simulink model "RADTRANS002"  (R2020b)
(part 2 of 7)

      |     % Цикл начинаем с 2, так как 1-й элемент в списке - это сама папка подсистемы
      |     for i = 2:length(internalBlocks)
      |         oldName = get_param(internalBlocks{i}, 'Name');
      |         % Ищем цифру в конце имени и меняем на новую
      |         newName = regexprep(oldName, '\d+$', newNum);
      | 
      |         % Если имя изменилось, применяем его
      |         if ~strcmp(oldName, newName)
      |             try
      |                 set_param(internalBlocks{i}, 'Name', newName);
      |             catch
      |                 % Игнорируем ошибку, если вдруг такое имя уже случайно есть
      |             end
      |         end
      |     end
      | end
  M_OUT_Завод_4_2 : Subsystem
      settings: CopyFcn=|
      | % Получаем путь и имя нового (только что скопированного) блока
      | blockPath = gcb;
      | blockName = get_param(blockPath, 'Name');
      | 
      | % Ищем число в названии самой подсистемы (например, берем "2" из "Measure_2")
      | numStr = regexp(blockName, '\d+', 'match');
      | 
      | if ~isempty(numStr)
      |     newNum = numStr{end}; % Берем последнее найденное число
      | 
      |     % --- 1. Обновляем скрытые теги в Goto и From (радиочастоты) ---
      |     gotos = find_system(blockPath, 'LookUnderMasks', 'on', 'BlockType', 'Goto');
      |     froms = find_system(blockPath, 'LookUnderMasks', 'on', 'BlockType', 'From');
      | 
      |     for i = 1:length(gotos)
      |         oldTag = get_param(gotos{i}, 'GotoTag');
      |         set_param(gotos{i}, 'GotoTag', regexprep(oldTag, '\d+$', newNum));
      |     end
      |     for i = 1:length(froms)
      |         oldTag = get_param(froms{i}, 'GotoTag');
      |         set_param(froms{i}, 'GotoTag', regexprep(oldTag, '\d+$', newNum));
      |     end
      | 
      |     % --- 2. ПЕРЕИМЕНОВЫВАЕМ САМИ БЛОКИ (визуальные надписи UI0 -> UI1 и т.д.) ---
      |     % Ищем все элементы только внутри этой подсистемы
      |     internalBlocks = find_system(blockPath, 'SearchDepth', 1, 'LookUnderMasks', 'on');
      | 
      |     % Цикл начинаем с 2, так как 1-й элемент в списке - это сама папка подсистемы
      |     for i = 2:length(internalBlocks)
      |         oldName = get_param(internalBlocks{i}, 'Name');
      |         % Ищем цифру в конце имени и меняем на новую
      |         newName = regexprep(oldName, '\d+$', newNum);
      | 
      |         % Если имя изменилось, применяем его
      |         if ~strcmp(oldName, newName)
      |             try
      |                 set_param(internalBlocks{i}, 'Name', newName);
      |             catch
      |                 % Игнорируем ошибку, если вдруг такое имя уже случайно есть
      |             end
      |         end
      |     end
      | end
  M_OUT_Завод_5_1 : Subsystem
      settings: CopyFcn=|
      | % Получаем путь и имя нового (только что скопированного) блока
      | blockPath = gcb;
      | blockName = get_param(blockPath, 'Name');
      | 
      | % Ищем число в названии самой подсистемы (например, берем "2" из "Measure_2")
      | numStr = regexp(blockName, '\d+', 'match');
      | 
      | if ~isempty(numStr)
      |     newNum = numStr{end}; % Берем последнее найденное число
      | 
      |     % --- 1. Обновляем скрытые теги в Goto и From (радиочастоты) ---
      |     gotos = find_system(blockPath, 'LookUnderMasks', 'on', 'BlockType', 'Goto');
      |     froms = find_system(blockPath, 'LookUnderMasks', 'on', 'BlockType', 'From');
      | 
      |     for i = 1:length(gotos)
      |         oldTag = get_param(gotos{i}, 'GotoTag');
      |         set_param(gotos{i}, 'GotoTag', regexprep(oldTag, '\d+$', newNum));
      |     end
      |     for i = 1:length(froms)
      |         oldTag = get_param(froms{i}, 'GotoTag');
      |         set_param(froms{i}, 'GotoTag', regexprep(oldTag, '\d+$', newNum));
      |     end
      | 
      |     % --- 2. ПЕРЕИМЕНОВЫВАЕМ САМИ БЛОКИ (визуальные надписи UI0 -> UI1 и т.д.) ---
      |     % Ищем все элементы только внутри этой подсистемы
      |     internalBlocks = find_system(blockPath, 'SearchDepth', 1, 'LookUnderMasks', 'on');
      | 
      |     % Цикл начинаем с 2, так как 1-й элемент в списке - это сама папка подсистемы
      |     for i = 2:length(internalBlocks)
      |         oldName = get_param(internalBlocks{i}, 'Name');
      |         % Ищем цифру в конце имени и меняем на новую
      |         newName = regexprep(oldName, '\d+$', newNum);
      | 
      |         % Если имя изменилось, применяем его
      |         if ~strcmp(oldName, newName)
      |             try
      |                 set_param(internalBlocks{i}, 'Name', newName);
      |             catch
      |                 % Игнорируем ошибку, если вдруг такое имя уже случайно есть
      |             end
      |         end
      |     end
      | end
  M_OUT_Завод_5_2 : Subsystem
      settings: CopyFcn=|
      | % Получаем путь и имя нового (только что скопированного) блока
      | blockPath = gcb;
      | blockName = get_param(blockPath, 'Name');
      | 
      | % Ищем число в названии самой подсистемы (например, берем "2" из "Measure_2")
      | numStr = regexp(blockName, '\d+', 'match');
      | 
      | if ~isempty(numStr)
      |     newNum = numStr{end}; % Берем последнее найденное число
      | 
      |     % --- 1. Обновляем скрытые теги в Goto и From (радиочастоты) ---
      |     gotos = find_system(blockPath, 'LookUnderMasks', 'on', 'BlockType', 'Goto');
      |     froms = find_system(blockPath, 'LookUnderMasks', 'on', 'BlockType', 'From');
      | 
      |     for i = 1:length(gotos)
      |         oldTag = get_param(gotos{i}, 'GotoTag');
      |         set_param(gotos{i}, 'GotoTag', regexprep(oldTag, '\d+$', newNum));
      |     end
      |     for i = 1:length(froms)
      |         oldTag = get_param(froms{i}, 'GotoTag');
      |         set_param(froms{i}, 'GotoTag', regexprep(oldTag, '\d+$', newNum));
      |     end
      | 
      |     % --- 2. ПЕРЕИМЕНОВЫВАЕМ САМИ БЛОКИ (визуальные надписи UI0 -> UI1 и т.д.) ---
      |     % Ищем все элементы только внутри этой подсистемы
      |     internalBlocks = find_system(blockPath, 'SearchDepth', 1, 'LookUnderMasks', 'on');
      | 
      |     % Цикл начинаем с 2, так как 1-й элемент в списке - это сама папка подсистемы
      |     for i = 2:length(internalBlocks)
      |         oldName = get_param(internalBlocks{i}, 'Name');
      |         % Ищем цифру в конце имени и меняем на новую
      |         newName = regexprep(oldName, '\d+$', newNum);
      | 
      |         % Если имя изменилось, применяем его
      |         if ~strcmp(oldName, newName)
      |             try
      |                 set_param(internalBlocks{i}, 'Name', newName);
      |             catch
      |                 % Игнорируем ошибку, если вдруг такое имя уже случайно есть
      |             end
      |         end
      |     end
      | end
  M_OUT_Завод_6_1 : Subsystem
      settings: CopyFcn=|
      | % Получаем путь и имя нового (только что скопированного) блока
      | blockPath = gcb;
      | blockName = get_param(blockPath, 'Name');
      | 
      | % Ищем число в названии самой подсистемы (например, берем "2" из "Measure_2")
      | numStr = regexp(blockName, '\d+', 'match');
      | 
      | if ~isempty(numStr)
      |     newNum = numStr{end}; % Берем последнее найденное число
      | 
      |     % --- 1. Обновляем скрытые теги в Goto и From (радиочастоты) ---
      |     gotos = find_system(blockPath, 'LookUnderMasks', 'on', 'BlockType', 'Goto');
      |     froms = find_system(blockPath, 'LookUnderMasks', 'on', 'BlockType', 'From');
      | 
      |     for i = 1:length(gotos)
      |         oldTag = get_param(gotos{i}, 'GotoTag');
      |         set_param(gotos{i}, 'GotoTag', regexprep(oldTag, '\d+$', newNum));
      |     end
      |     for i = 1:length(froms)
      |         oldTag = get_param(froms{i}, 'GotoTag');
      |         set_param(froms{i}, 'GotoTag', regexprep(oldTag, '\d+$', newNum));
      |     end
      | 
      |     % --- 2. ПЕРЕИМЕНОВЫВАЕМ САМИ БЛОКИ (визуальные надписи UI0 -> UI1 и т.д.) ---
      |     % Ищем все элементы только внутри этой подсистемы
      |     internalBlocks = find_system(blockPath, 'SearchDepth', 1, 'LookUnderMasks', 'on');
      | 
      |     % Цикл начинаем с 2, так как 1-й элемент в списке - это сама папка подсистемы
      |     for i = 2:length(internalBlocks)
      |         oldName = get_param(internalBlocks{i}, 'Name');
      |         % Ищем цифру в конце имени и меняем на новую
      |         newName = regexprep(oldName, '\d+$', newNum);
      | 
      |         % Если имя изменилось, применяем его
      |         if ~strcmp(oldName, newName)
      |             try
      |                 set_param(internalBlocks{i}, 'Name', newName);
      |             catch
      |                 % Игнорируем ошибку, если вдруг такое имя уже случайно есть
      |             end
      |         end
      |     end
      | end
  M_OUT_Завод_6_2 : Subsystem
      settings: CopyFcn=|
      | % Получаем путь и имя нового (только что скопированного) блока
      | blockPath = gcb;
      | blockName = get_param(blockPath, 'Name');
      | 
      | % Ищем число в названии самой подсистемы (например, берем "2" из "Measure_2")
      | numStr = regexp(blockName, '\d+', 'match');
      | 
      | if ~isempty(numStr)
      |     newNum = numStr{end}; % Берем последнее найденное число
      | 
      |     % --- 1. Обновляем скрытые теги в Goto и From (радиочастоты) ---
      |     gotos = find_system(blockPath, 'LookUnderMasks', 'on', 'BlockType', 'Goto');
      |     froms = find_system(blockPath, 'LookUnderMasks', 'on', 'BlockType', 'From');
      | 
      |     for i = 1:length(gotos)
      |         oldTag = get_param(gotos{i}, 'GotoTag');
      |         set_param(gotos{i}, 'GotoTag', regexprep(oldTag, '\d+$', newNum));
      |     end
      |     for i = 1:length(froms)
      |         oldTag = get_param(froms{i}, 'GotoTag');
      |         set_param(froms{i}, 'GotoTag', regexprep(oldTag, '\d+$', newNum));
      |     end
      | 
      |     % --- 2. ПЕРЕИМЕНОВЫВАЕМ САМИ БЛОКИ (визуальные надписи UI0 -> UI1 и т.д.) ---
      |     % Ищем все элементы только внутри этой подсистемы
      |     internalBlocks = find_system(blockPath, 'SearchDepth', 1, 'LookUnderMasks', 'on');
      | 
      |     % Цикл начинаем с 2, так как 1-й элемент в списке - это сама папка подсистемы
      |     for i = 2:length(internalBlocks)
      |         oldName = get_param(internalBlocks{i}, 'Name');
      |         % Ищем цифру в конце имени и меняем на новую
      |         newName = regexprep(oldName, '\d+$', newNum);
      | 
      |         % Если имя изменилось, применяем его
      |         if ~strcmp(oldName, newName)
      |             try
      |                 set_param(internalBlocks{i}, 'Name', newName);
      |             catch
      |                 % Игнорируем ошибку, если вдруг такое имя уже случайно есть
      |             end
      |         end
      |     end
      | end
  Powergui : powerlib/powergui  Priority=1  SimulationMode=Discrete  SampleTime=Ts_powergui  frequency=60  Iterations=50  frequencyindice=50  Pbase=100e6  ErrMax=1e-4  UnitsV=kV  UnitsW=MW  buscounter=0  FunctionMessages=off  echomessages=off  EnableUseOfTLC=off  CurrentSourceSwitches=off  DisableSnubberDevices=off  DisableRonSwitches=off  DisableVfSwitches=off  DisplayEquations=off  AutomaticDiscreteSolvers=off  SolverType=Tustin/Backward Euler (TBE)  Interpol=off  ExternalGateDelay=off  methode=off  Ts=100  x0status=blocks  SPID=on  SwTol=0  HookPort=off  NonlinearTolerance=1e-4  nMaxIteration=100  ContinueOnMaxIteration=off  RestoreLinks=warning  ResistiveCurrentMeasurement=off  Frange=[0:2:500]  Ylog=off  Xlog=on  ShowGrid=off  save=off  variable=ZData  structure=0  ZoomFFT=off  StartTime=0.0  cycles=1  DisplayStyle=1  fundamental=60  FreqAxis=off  MaxFrequency=1000  frequencyindicesteady=1  RmsSteady=1  display=off
  Источник_220кВ : powerlib/Electrical Sources/Three-Phase Source  InternalConnection=Yg  VoltagePhases=off  Voltage=Sys_V_net_kV * 1e3  PhaseAngle=0  Voltage_phases=[25e3 25e3 25e3]/sqrt(3)  PhaseAngles_phases=[0 -120 +120]  Frequency=Sys_f_Hz  NonIdealSource=on  SpecifyImpedance=off  Resistance=0.8929  Inductance=16.58e-3  ShortCircuitLevel=Sys_S_sc_VA  BaseVoltage=Sys_V_net_kV * 1e3  XRratio=7  BusType=swing  Pref=10e3  Qref=0  Prefabc=[10e3, 10e3, 10e3]  Qrefabc=[0, 0, 0]  Qmin=-inf  Qmax=inf
  Линия_110кВ_Район_{1..6} (6 alike) : powerlib/Elements/Three-Phase PI Section Line  LConnTagsString=a|b|c  RConnTagsString=A|B|C  Length=1  Frequency=Sys_f_Hz  Resistances=[Line_110_R, Line_110_R*3]  Inductances=[Line_110_L, Line_110_L*3]  Capacitances=[Line_110_C, Line_110_C]
  Линия_Город_1_{1..4} (4 alike) : powerlib/Elements/Three-Phase PI Section Line  LConnTagsString=a|b|c  RConnTagsString=A|B|C  Length=1  Frequency=Sys_f_Hz  Resistances=[Line_6_R, Line_6_R*3]  Inductances=[Line_6_L, Line_6_L*3]  Capacitances=[1e-9, 1e-9]
  Линия_Город_2_{1..4} (4 alike) : powerlib/Elements/Three-Phase PI Section Line  LConnTagsString=a|b|c  RConnTagsString=A|B|C  Length=1  Frequency=Sys_f_Hz  Resistances=[Line_6_R, Line_6_R*3]  Inductances=[Line_6_L, Line_6_L*3]  Capacitances=[1e-9, 1e-9]
  Линия_Город_3_{1..4} (4 alike) : powerlib/Elements/Three-Phase PI Section Line  LConnTagsString=a|b|c  RConnTagsString=A|B|C  Length=1  Frequency=Sys_f_Hz  Resistances=[Line_6_R, Line_6_R*3]  Inductances=[Line_6_L, Line_6_L*3]  Capacitances=[1e-9, 1e-9]
  Линия_Город_4_{1..4} (4 alike) : powerlib/Elements/Three-Phase PI Section Line  LConnTagsString=a|b|c  RConnTagsString=A|B|C  Length=1  Frequency=Sys_f_Hz  Resistances=[Line_6_R, Line_6_R*3]  Inductances=[Line_6_L, Line_6_L*3]  Capacitances=[1e-9, 1e-9]
  Линия_Город_5_{1..4} (4 alike) : powerlib/Elements/Three-Phase PI Section Line  LConnTagsString=a|b|c  RConnTagsString=A|B|C  Length=1  Frequency=Sys_f_Hz  Resistances=[Line_6_R, Line_6_R*3]  Inductances=[Line_6_L, Line_6_L*3]  Capacitances=[1e-9, 1e-9]
  Линия_Город_6_{1..4} (4 alike) : powerlib/Elements/Three-Phase PI Section Line  LConnTagsString=a|b|c  RConnTagsString=A|B|C  Length=1  Frequency=Sys_f_Hz  Resistances=[Line_6_R, Line_6_R*3]  Inductances=[Line_6_L, Line_6_L*3]  Capacitances=[1e-9, 1e-9]
  Линия_Завод_1_1 : powerlib/Elements/Three-Phase PI Section Line  LConnTagsString=a|b|c  RConnTagsString=A|B|C  Length=1  Frequency=Sys_f_Hz  Resistances=[Line_35_R, Line_35_R*3]  Inductances=[Line_35_L, Line_35_L*3]  Capacitances=[Line_35_C, Line_35_C]
  Линия_Завод_1_2 : powerlib/Elements/Three-Phase PI Section Line  LConnTagsString=a|b|c  RConnTagsString=A|B|C  Length=1  Frequency=Sys_f_Hz  Resistances=[Line_35_R, Line_35_R*3]  Inductances=[Line_35_L, Line_35_L*3]  Capacitances=[Line_35_C, Line_35_C]
  Линия_Завод_2_1 : powerlib/Elements/Three-Phase PI Section Line  LConnTagsString=a|b|c  RConnTagsString=A|B|C  Length=1  Frequency=Sys_f_Hz  Resistances=[Line_35_R, Line_35_R*3]  Inductances=[Line_35_L, Line_35_L*3]  Capacitances=[Line_35_C, Line_35_C]
  Линия_Завод_2_2 : powerlib/Elements/Three-Phase PI Section Line  LConnTagsString=a|b|c  RConnTagsString=A|B|C  Length=1  Frequency=Sys_f_Hz  Resistances=[Line_35_R, Line_35_R*3]  Inductances=[Line_35_L, Line_35_L*3]  Capacitances=[Line_35_C, Line_35_C]
  Линия_Завод_3_1 : powerlib/Elements/Three-Phase PI Section Line  LConnTagsString=a|b|c  RConnTagsString=A|B|C  Length=1  Frequency=Sys_f_Hz  Resistances=[Line_35_R, Line_35_R*3]  Inductances=[Line_35_L, Line_35_L*3]  Capacitances=[Line_35_C, Line_35_C]
  Линия_Завод_3_2 : powerlib/Elements/Three-Phase PI Section Line  LConnTagsString=a|b|c  RConnTagsString=A|B|C  Length=1  Frequency=Sys_f_Hz  Resistances=[Line_35_R, Line_35_R*3]  Inductances=[Line_35_L, Line_35_L*3]  Capacitances=[Line_35_C, Line_35_C]
  Линия_Завод_4_1 : powerlib/Elements/Three-Phase PI Section Line  LConnTagsString=a|b|c  RConnTagsString=A|B|C  Length=1  Frequency=Sys_f_Hz  Resistances=[Line_35_R, Line_35_R*3]  Inductances=[Line_35_L, Line_35_L*3]  Capacitances=[Line_35_C, Line_35_C]
  Линия_Завод_4_2 : powerlib/Elements/Three-Phase PI Section Line  LConnTagsString=a|b|c  RConnTagsString=A|B|C  Length=1  Frequency=Sys_f_Hz  Resistances=[Line_35_R, Line_35_R*3]  Inductances=[Line_35_L, Line_35_L*3]  Capacitances=[Line_35_C, Line_35_C]
  Линия_Завод_5_1 : powerlib/Elements/Three-Phase PI Section Line  LConnTagsString=a|b|c  RConnTagsString=A|B|C  Length=1  Frequency=Sys_f_Hz  Resistances=[Line_35_R, Line_35_R*3]  Inductances=[Line_35_L, Line_35_L*3]  Capacitances=[Line_35_C, Line_35_C]
  Линия_Завод_5_2 : powerlib/Elements/Three-Phase PI Section Line  LConnTagsString=a|b|c  RConnTagsString=A|B|C  Length=1  Frequency=Sys_f_Hz  Resistances=[Line_35_R, Line_35_R*3]  Inductances=[Line_35_L, Line_35_L*3]  Capacitances=[Line_35_C, Line_35_C]
  Линия_Завод_6_1 : powerlib/Elements/Three-Phase PI Section Line  LConnTagsString=a|b|c  RConnTagsString=A|B|C  Length=1  Frequency=Sys_f_Hz  Resistances=[Line_35_R, Line_35_R*3]  Inductances=[Line_35_L, Line_35_L*3]  Capacitances=[Line_35_C, Line_35_C]
  Линия_Завод_6_2 : powerlib/Elements/Three-Phase PI Section Line  LConnTagsString=a|b|c  RConnTagsString=A|B|C  Length=1  Frequency=Sys_f_Hz  Resistances=[Line_35_R, Line_35_R*3]  Inductances=[Line_35_L, Line_35_L*3]  Capacitances=[Line_35_C, Line_35_C]
  Магистраль_220кВ : powerlib/Elements/Three-Phase PI Section Line  LConnTagsString=a|b|c  RConnTagsString=A|B|C  Length=1  Frequency=Sys_f_Hz  Resistances=[Line_220_R, Line_220_R*3]  Inductances=[Line_220_L, Line_220_L*3]  Capacitances=[Line_220_C, Line_220_C]
  Нагрузка_Город_1_{1..4} (4 alike) : powerlib/Elements/Three-Phase Series RLC Load  LConnTagsString=A|B|C  Configuration=Y (grounded)  NominalVoltage=Tr_6_04_V_LV_kV*1e3  Vabc=[1e3 1e3 1e3]  Vabcp=[1e3 1e3 1e3]  NominalFrequency=Sys_f_Hz  UnbalancedPower=off  ActivePower=Load_City_P  InductivePower=Load_City_Q  CapacitivePower=0  Pabc=[10e3 9e3 11e3]  QLabc=[100 90 110]  QCabc=[100 90 110]  Pabcp=[10e3 9e3 11e3]  QLabcp=[100 90 110]  QCabcp=[100 90 110]  Measurements=None  LoadType=constant Z
  Нагрузка_Город_2_{1..4} (4 alike) : powerlib/Elements/Three-Phase Series RLC Load  LConnTagsString=A|B|C  Configuration=Y (grounded)  NominalVoltage=Tr_6_04_V_LV_kV*1e3  Vabc=[1e3 1e3 1e3]  Vabcp=[1e3 1e3 1e3]  NominalFrequency=Sys_f_Hz  UnbalancedPower=off  ActivePower=Load_City_P  InductivePower=Load_City_Q  CapacitivePower=0  Pabc=[10e3 9e3 11e3]  QLabc=[100 90 110]  QCabc=[100 90 110]  Pabcp=[10e3 9e3 11e3]  QLabcp=[100 90 110]  QCabcp=[100 90 110]  Measurements=None  LoadType=constant Z
  Нагрузка_Город_3_{1..4} (4 alike) : powerlib/Elements/Three-Phase Series RLC Load  LConnTagsString=A|B|C  Configuration=Y (grounded)  NominalVoltage=Tr_6_04_V_LV_kV*1e3  Vabc=[1e3 1e3 1e3]  Vabcp=[1e3 1e3 1e3]  NominalFrequency=Sys_f_Hz  UnbalancedPower=off  ActivePower=Load_City_P  InductivePower=Load_City_Q  CapacitivePower=0  Pabc=[10e3 9e3 11e3]  QLabc=[100 90 110]  QCabc=[100 90 110]  Pabcp=[10e3 9e3 11e3]  QLabcp=[100 90 110]  QCabcp=[100 90 110]  Measurements=None  LoadType=constant Z
  Нагрузка_Город_4_{1..4} (4 alike) : powerlib/Elements/Three-Phase Series RLC Load  LConnTagsString=A|B|C  Configuration=Y (grounded)  NominalVoltage=Tr_6_04_V_LV_kV*1e3  Vabc=[1e3 1e3 1e3]  Vabcp=[1e3 1e3 1e3]  NominalFrequency=Sys_f_Hz  UnbalancedPower=off  ActivePower=Load_City_P  InductivePower=Load_City_Q  CapacitivePower=0  Pabc=[10e3 9e3 11e3]  QLabc=[100 90 110]  QCabc=[100 90 110]  Pabcp=[10e3 9e3 11e3]  QLabcp=[100 90 110]  QCabcp=[100 90 110]  Measurements=None  LoadType=constant Z
  Нагрузка_Город_5_{1..4} (4 alike) : powerlib/Elements/Three-Phase Series RLC Load  LConnTagsString=A|B|C  Configuration=Y (grounded)  NominalVoltage=Tr_6_04_V_LV_kV*1e3  Vabc=[1e3 1e3 1e3]  Vabcp=[1e3 1e3 1e3]  NominalFrequency=Sys_f_Hz  UnbalancedPower=off  ActivePower=Load_City_P  InductivePower=Load_City_Q  CapacitivePower=0  Pabc=[10e3 9e3 11e3]  QLabc=[100 90 110]  QCabc=[100 90 110]  Pabcp=[10e3 9e3 11e3]  QLabcp=[100 90 110]  QCabcp=[100 90 110]  Measurements=None  LoadType=constant Z
  Нагрузка_Город_6_{1..4} (4 alike) : powerlib/Elements/Three-Phase Series RLC Load  LConnTagsString=A|B|C  Configuration=Y (grounded)  NominalVoltage=Tr_6_04_V_LV_kV*1e3  Vabc=[1e3 1e3 1e3]  Vabcp=[1e3 1e3 1e3]  NominalFrequency=Sys_f_Hz  UnbalancedPower=off  ActivePower=Load_City_P  InductivePower=Load_City_Q  CapacitivePower=0  Pabc=[10e3 9e3 11e3]  QLabc=[100 90 110]  QCabc=[100 90 110]  Pabcp=[10e3 9e3 11e3]  QLabcp=[100 90 110]  QCabcp=[100 90 110]  Measurements=None  LoadType=constant Z
  Нагрузка_Завод_1_1 : powerlib/Elements/Three-Phase Series RLC Load  LConnTagsString=A|B|C  Configuration=Y (grounded)  NominalVoltage=Tr_35_04_V_LV_kV*1e3  Vabc=[1e3 1e3 1e3]  Vabcp=[1e3 1e3 1e3]  NominalFrequency=Sys_f_Hz  UnbalancedPower=off  ActivePower=Load_Factory_P  InductivePower=Load_Factory_Q  CapacitivePower=0  Pabc=[10e3 9e3 11e3]  QLabc=[100 90 110]  QCabc=[100 90 110]  Pabcp=[10e3 9e3 11e3]  QLabcp=[100 90 110]  QCabcp=[100 90 110]  Measurements=None  LoadType=constant Z
  Нагрузка_Завод_1_2 : powerlib/Elements/Three-Phase Series RLC Load  LConnTagsString=A|B|C  Configuration=Y (grounded)  NominalVoltage=Tr_35_04_V_LV_kV*1e3  Vabc=[1e3 1e3 1e3]  Vabcp=[1e3 1e3 1e3]  NominalFrequency=Sys_f_Hz  UnbalancedPower=off  ActivePower=Load_Factory_P  InductivePower=Load_Factory_Q  CapacitivePower=0  Pabc=[10e3 9e3 11e3]  QLabc=[100 90 110]  QCabc=[100 90 110]  Pabcp=[10e3 9e3 11e3]  QLabcp=[100 90 110]  QCabcp=[100 90 110]  Measurements=None  LoadType=constant Z
  Нагрузка_Завод_2_1 : powerlib/Elements/Three-Phase Series RLC Load  LConnTagsString=A|B|C  Configuration=Y (grounded)  NominalVoltage=Tr_35_04_V_LV_kV*1e3  Vabc=[1e3 1e3 1e3]  Vabcp=[1e3 1e3 1e3]  NominalFrequency=Sys_f_Hz  UnbalancedPower=off  ActivePower=Load_Factory_P  InductivePower=Load_Factory_Q  CapacitivePower=0  Pabc=[10e3 9e3 11e3]  QLabc=[100 90 110]  QCabc=[100 90 110]  Pabcp=[10e3 9e3 11e3]  QLabcp=[100 90 110]  QCabcp=[100 90 110]  Measurements=None  LoadType=constant Z
  Нагрузка_Завод_2_2 : powerlib/Elements/Three-Phase Series RLC Load  LConnTagsString=A|B|C  Configuration=Y (grounded)  NominalVoltage=Tr_35_04_V_LV_kV*1e3  Vabc=[1e3 1e3 1e3]  Vabcp=[1e3 1e3 1e3]  NominalFrequency=Sys_f_Hz  UnbalancedPower=off  ActivePower=Load_Factory_P  InductivePower=Load_Factory_Q  CapacitivePower=0  Pabc=[10e3 9e3 11e3]  QLabc=[100 90 110]  QCabc=[100 90 110]  Pabcp=[10e3 9e3 11e3]  QLabcp=[100 90 110]  QCabcp=[100 90 110]  Measurements=None  LoadType=constant Z
  Нагрузка_Завод_3_1 : powerlib/Elements/Three-Phase Series RLC Load  LConnTagsString=A|B|C  Configuration=Y (grounded)  NominalVoltage=Tr_35_04_V_LV_kV*1e3  Vabc=[1e3 1e3 1e3]  Vabcp=[1e3 1e3 1e3]  NominalFrequency=Sys_f_Hz  UnbalancedPower=off  ActivePower=Load_Factory_P  InductivePower=Load_Factory_Q  CapacitivePower=0  Pabc=[10e3 9e3 11e3]  QLabc=[100 90 110]  QCabc=[100 90 110]  Pabcp=[10e3 9e3 11e3]  QLabcp=[100 90 110]  QCabcp=[100 90 110]  Measurements=None  LoadType=constant Z
  Нагрузка_Завод_3_2 : powerlib/Elements/Three-Phase Series RLC Load  LConnTagsString=A|B|C  Configuration=Y (grounded)  NominalVoltage=Tr_35_04_V_LV_kV*1e3  Vabc=[1e3 1e3 1e3]  Vabcp=[1e3 1e3 1e3]  NominalFrequency=Sys_f_Hz  UnbalancedPower=off  ActivePower=Load_Factory_P  InductivePower=Load_Factory_Q  CapacitivePower=0  Pabc=[10e3 9e3 11e3]  QLabc=[100 90 110]  QCabc=[100 90 110]  Pabcp=[10e3 9e3 11e3]  QLabcp=[100 90 110]  QCabcp=[100 90 110]  Measurements=None  LoadType=constant Z
  Нагрузка_Завод_4_1 : powerlib/Elements/Three-Phase Series RLC Load  LConnTagsString=A|B|C  Configuration=Y (grounded)  NominalVoltage=Tr_35_04_V_LV_kV*1e3  Vabc=[1e3 1e3 1e3]  Vabcp=[1e3 1e3 1e3]  NominalFrequency=Sys_f_Hz  UnbalancedPower=off  ActivePower=Load_Factory_P  InductivePower=Load_Factory_Q  CapacitivePower=0  Pabc=[10e3 9e3 11e3]  QLabc=[100 90 110]  QCabc=[100 90 110]  Pabcp=[10e3 9e3 11e3]  QLabcp=[100 90 110]  QCabcp=[100 90 110]  Measurements=None  LoadType=constant Z
  Нагрузка_Завод_4_2 : powerlib/Elements/Three-Phase Series RLC Load  LConnTagsString=A|B|C  Configuration=Y (grounded)  NominalVoltage=Tr_35_04_V_LV_kV*1e3  Vabc=[1e3 1e3 1e3]  Vabcp=[1e3 1e3 1e3]  NominalFrequency=Sys_f_Hz  UnbalancedPower=off  ActivePower=Load_Factory_P  InductivePower=Load_Factory_Q  CapacitivePower=0  Pabc=[10e3 9e3 11e3]  QLabc=[100 90 110]  QCabc=[100 90 110]  Pabcp=[10e3 9e3 11e3]  QLabcp=[100 90 110]  QCabcp=[100 90 110]  Measurements=None  LoadType=constant Z
  Нагрузка_Завод_5_1 : powerlib/Elements/Three-Phase Series RLC Load  LConnTagsString=A|B|C  Configuration=Y (grounded)  NominalVoltage=Tr_35_04_V_LV_kV*1e3  Vabc=[1e3 1e3 1e3]  Vabcp=[1e3 1e3 1e3]  NominalFrequency=Sys_f_Hz  UnbalancedPower=off  ActivePower=Load_Factory_P  InductivePower=Load_Factory_Q  CapacitivePower=0  Pabc=[10e3 9e3 11e3]  QLabc=[100 90 110]  QCabc=[100 90 110]  Pabcp=[10e3 9e3 11e3]  QLabcp=[100 90 110]  QCabcp=[100 90 110]  Measurements=None  LoadType=constant Z
  Нагрузка_Завод_5_2 : powerlib/Elements/Three-Phase Series RLC Load  LConnTagsString=A|B|C  Configuration=Y (grounded)  NominalVoltage=Tr_35_04_V_LV_kV*1e3  Vabc=[1e3 1e3 1e3]  Vabcp=[1e3 1e3 1e3]  NominalFrequency=Sys_f_Hz  UnbalancedPower=off  ActivePower=Load_Factory_P  InductivePower=Load_Factory_Q  CapacitivePower=0  Pabc=[10e3 9e3 11e3]  QLabc=[100 90 110]  QCabc=[100 90 110]  Pabcp=[10e3 9e3 11e3]  QLabcp=[100 90 110]  QCabcp=[100 90 110]  Measurements=None  LoadType=constant Z
  Нагрузка_Завод_6_1 : powerlib/Elements/Three-Phase Series RLC Load  LConnTagsString=A|B|C  Configuration=Y (grounded)  NominalVoltage=Tr_35_04_V_LV_kV*1e3  Vabc=[1e3 1e3 1e3]  Vabcp=[1e3 1e3 1e3]  NominalFrequency=Sys_f_Hz  UnbalancedPower=off  ActivePower=Load_Factory_P  InductivePower=Load_Factory_Q  CapacitivePower=0  Pabc=[10e3 9e3 11e3]  QLabc=[100 90 110]  QCabc=[100 90 110]  Pabcp=[10e3 9e3 11e3]  QLabcp=[100 90 110]  QCabcp=[100 90 110]  Measurements=None  LoadType=constant Z
  Нагрузка_Завод_6_2 : powerlib/Elements/Three-Phase Series RLC Load  LConnTagsString=A|B|C  Configuration=Y (grounded)  NominalVoltage=Tr_35_04_V_LV_kV*1e3  Vabc=[1e3 1e3 1e3]  Vabcp=[1e3 1e3 1e3]  NominalFrequency=Sys_f_Hz  UnbalancedPower=off  ActivePower=Load_Factory_P  InductivePower=Load_Factory_Q  CapacitivePower=0  Pabc=[10e3 9e3 11e3]  QLabc=[100 90 110]  QCabc=[100 90 110]  Pabcp=[10e3 9e3 11e3]  QLabcp=[100 90 110]  QCabcp=[100 90 110]  Measurements=None  LoadType=constant Z
  Трансформатор_110_35_Район_{1..6} (6 alike) : powerlib/Elements/Three-Phase Transformer (Two Windings)  Winding1Connection=Yg  Winding2Connection=Yg  CoreType=Three single-phase transformers  SetSaturation=off  Hysteresis=off  DataFile='hysteresis'  SetInitialFlux=off  Measurements=None  UNITS=pu  NominalPower=[Tr_110_35_Sn_VA, Sys_f_Hz]  Winding1=[Tr_110_35_V_HV_kV*1e3, Tr_110_35_R_pu, Tr_110_35_L_pu]  Winding2=[Tr_110_35_V_LV_kV*1e3, Tr_110_35_R_pu, Tr_110_35_L_pu]  Rm=500  Lm=500  L0=0.5  Saturation=[ 0,0 ; 0.0024,1.2 ; 1.0,1.52 ]  InitialFluxes=[ 0.8 , -0.8 , 0.7 ]  BreakLoop=off  DiscreteSolver=Trapezoidal iterative  DataType=off  TransfoNumber=1
  Трансформатор_110_6_Район_{1..6} (6 alike) : powerlib/Elements/Three-Phase Transformer (Two Windings)  Winding1Connection=Yg  Winding2Connection=Yg  CoreType=Three single-phase transformers  SetSaturation=off  Hysteresis=off  DataFile='hysteresis'  SetInitialFlux=off  Measurements=None  UNITS=pu  NominalPower=[Tr_110_6_Sn_VA, Sys_f_Hz]  Winding1=[Tr_110_6_V_HV_kV*1e3, Tr_110_6_R_pu, Tr_110_6_L_pu]  Winding2=[Tr_110_6_V_LV_kV*1e3, Tr_110_6_R_pu, Tr_110_6_L_pu]  Rm=500  Lm=500  L0=0.5  Saturation=[ 0,0 ; 0.0024,1.2 ; 1.0,1.52 ]  InitialFluxes=[ 0.8 , -0.8 , 0.7 ]  BreakLoop=off  DiscreteSolver=Trapezoidal iterative  DataType=off  TransfoNumber=1
  Трансформатор_Город_1_{1..4} (4 alike) : powerlib/Elements/Three-Phase Transformer (Two Windings)  Winding1Connection=Yg  Winding2Connection=Yg  CoreType=Three single-phase transformers  SetSaturation=off  Hysteresis=off  DataFile='hysteresis'  SetInitialFlux=off  Measurements=None  UNITS=pu  NominalPower=[Tr_6_04_Sn_VA, Sys_f_Hz]  Winding1=[Tr_6_04_V_HV_kV*1e3, Tr_6_04_R_pu, Tr_6_04_L_pu]  Winding2=[Tr_6_04_V_LV_kV*1e3, Tr_6_04_R_pu, Tr_6_04_L_pu]  Rm=500  Lm=500  L0=0.5  Saturation=[ 0,0 ; 0.0024,1.2 ; 1.0,1.52 ]  InitialFluxes=[ 0.8 , -0.8 , 0.7 ]  BreakLoop=off  DiscreteSolver=Trapezoidal iterative  DataType=off  TransfoNumber=1
  Трансформатор_Город_2_{1..4} (4 alike) : powerlib/Elements/Three-Phase Transformer (Two Windings)  Winding1Connection=Yg  Winding2Connection=Yg  CoreType=Three single-phase transformers  SetSaturation=off  Hysteresis=off  DataFile='hysteresis'  SetInitialFlux=off  Measurements=None  UNITS=pu  NominalPower=[Tr_6_04_Sn_VA, Sys_f_Hz]  Winding1=[Tr_6_04_V_HV_kV*1e3, Tr_6_04_R_pu, Tr_6_04_L_pu]  Winding2=[Tr_6_04_V_LV_kV*1e3, Tr_6_04_R_pu, Tr_6_04_L_pu]  Rm=500  Lm=500  L0=0.5  Saturation=[ 0,0 ; 0.0024,1.2 ; 1.0,1.52 ]  InitialFluxes=[ 0.8 , -0.8 , 0.7 ]  BreakLoop=off  DiscreteSolver=Trapezoidal iterative  DataType=off  TransfoNumber=1
  Трансформатор_Город_3_{1..4} (4 alike) : powerlib/Elements/Three-Phase Transformer (Two Windings)  Winding1Connection=Yg  Winding2Connection=Yg  CoreType=Three single-phase transformers  SetSaturation=off  Hysteresis=off  DataFile='hysteresis'  SetInitialFlux=off  Measurements=None  UNITS=pu  NominalPower=[Tr_6_04_Sn_VA, Sys_f_Hz]  Winding1=[Tr_6_04_V_HV_kV*1e3, Tr_6_04_R_pu, Tr_6_04_L_pu]  Winding2=[Tr_6_04_V_LV_kV*1e3, Tr_6_04_R_pu, Tr_6_04_L_pu]  Rm=500  Lm=500  L0=0.5  Saturation=[ 0,0 ; 0.0024,1.2 ; 1.0,1.52 ]  InitialFluxes=[ 0.8 , -0.8 , 0.7 ]  BreakLoop=off  DiscreteSolver=Trapezoidal iterative  DataType=off  TransfoNumber=1
  Трансформатор_Город_4_{1..4} (4 alike) : powerlib/Elements/Three-Phase Transformer (Two Windings)  Winding1Connection=Yg  Winding2Connection=Yg  CoreType=Three single-phase transformers  SetSaturation=off  Hysteresis=off  DataFile='hysteresis'  SetInitialFlux=off  Measurements=None  UNITS=pu  NominalPower=[Tr_6_04_Sn_VA, Sys_f_Hz]  Winding1=[Tr_6_04_V_HV_kV*1e3, Tr_6_04_R_pu, Tr_6_04_L_pu]  Winding2=[Tr_6_04_V_LV_kV*1e3, Tr_6_04_R_pu, Tr_6_04_L_pu]  Rm=500  Lm=500  L0=0.5  Saturation=[ 0,0 ; 0.0024,1.2 ; 1.0,1.52 ]  InitialFluxes=[ 0.8 , -0.8 , 0.7 ]  BreakLoop=off  DiscreteSolver=Trapezoidal iterative  DataType=off  TransfoNumber=1
  Трансформатор_Город_5_{1..4} (4 alike) : powerlib/Elements/Three-Phase Transformer (Two Windings)  Winding1Connection=Yg  Winding2Connection=Yg  CoreType=Three single-phase transformers  SetSaturation=off  Hysteresis=off  DataFile='hysteresis'  SetInitialFlux=off  Measurements=None  UNITS=pu  NominalPower=[Tr_6_04_Sn_VA, Sys_f_Hz]  Winding1=[Tr_6_04_V_HV_kV*1e3, Tr_6_04_R_pu, Tr_6_04_L_pu]  Winding2=[Tr_6_04_V_LV_kV*1e3, Tr_6_04_R_pu, Tr_6_04_L_pu]  Rm=500  Lm=500  L0=0.5  Saturation=[ 0,0 ; 0.0024,1.2 ; 1.0,1.52 ]  InitialFluxes=[ 0.8 , -0.8 , 0.7 ]  BreakLoop=off  DiscreteSolver=Trapezoidal iterative  DataType=off  TransfoNumber=1
  Трансформатор_Город_6_{1..4} (4 alike) : powerlib/Elements/Three-Phase Transformer (Two Windings)  Winding1Connection=Yg  Winding2Connection=Yg  CoreType=Three single-phase transformers  SetSaturation=off  Hysteresis=off  DataFile='hysteresis'  SetInitialFlux=off  Measurements=None  UNITS=pu  NominalPower=[Tr_6_04_Sn_VA, Sys_f_Hz]  Winding1=[Tr_6_04_V_HV_kV*1e3, Tr_6_04_R_pu, Tr_6_04_L_pu]  Winding2=[Tr_6_04_V_LV_kV*1e3, Tr_6_04_R_pu, Tr_6_04_L_pu]  Rm=500  Lm=500  L0=0.5  Saturation=[ 0,0 ; 0.0024,1.2 ; 1.0,1.52 ]  InitialFluxes=[ 0.8 , -0.8 , 0.7 ]  BreakLoop=off  DiscreteSolver=Trapezoidal iterative  DataType=off  TransfoNumber=1
  Трансформатор_Завод_1_1 : powerlib/Elements/Three-Phase Transformer (Two Windings)  Winding1Connection=Yg  Winding2Connection=Yg  CoreType=Three single-phase transformers  SetSaturation=off  Hysteresis=off  DataFile='hysteresis'  SetInitialFlux=off  Measurements=None  UNITS=pu  NominalPower=[Tr_35_04_Sn_VA, Sys_f_Hz]  Winding1=[Tr_35_04_V_HV_kV*1e3, Tr_35_04_R_pu, Tr_35_04_L_pu]  Winding2=[Tr_35_04_V_LV_kV*1e3, Tr_35_04_R_pu, Tr_35_04_L_pu]  Rm=500  Lm=500  L0=0.5  Saturation=[ 0,0 ; 0.0024,1.2 ; 1.0,1.52 ]  InitialFluxes=[ 0.8 , -0.8 , 0.7 ]  BreakLoop=off  DiscreteSolver=Trapezoidal iterative  DataType=off  TransfoNumber=1
  Трансформатор_Завод_1_2 : powerlib/Elements/Three-Phase Transformer (Two Windings)  Winding1Connection=Yg  Winding2Connection=Yg  CoreType=Three single-phase transformers  SetSaturation=off  Hysteresis=off  DataFile='hysteresis'  SetInitialFlux=off  Measurements=None  UNITS=pu  NominalPower=[Tr_35_04_Sn_VA, Sys_f_Hz]  Winding1=[Tr_35_04_V_HV_kV*1e3, Tr_35_04_R_pu, Tr_35_04_L_pu]  Winding2=[Tr_35_04_V_LV_kV*1e3, Tr_35_04_R_pu, Tr_35_04_L_pu]  Rm=500  Lm=500  L0=0.5  Saturation=[ 0,0 ; 0.0024,1.2 ; 1.0,1.52 ]  InitialFluxes=[ 0.8 , -0.8 , 0.7 ]  BreakLoop=off  DiscreteSolver=Trapezoidal iterative  DataType=off  TransfoNumber=1
  Трансформатор_Завод_2_1 : powerlib/Elements/Three-Phase Transformer (Two Windings)  Winding1Connection=Yg  Winding2Connection=Yg  CoreType=Three single-phase transformers  SetSaturation=off  Hysteresis=off  DataFile='hysteresis'  SetInitialFlux=off  Measurements=None  UNITS=pu  NominalPower=[Tr_35_04_Sn_VA, Sys_f_Hz]  Winding1=[Tr_35_04_V_HV_kV*1e3, Tr_35_04_R_pu, Tr_35_04_L_pu]  Winding2=[Tr_35_04_V_LV_kV*1e3, Tr_35_04_R_pu, Tr_35_04_L_pu]  Rm=500  Lm=500  L0=0.5  Saturation=[ 0,0 ; 0.0024,1.2 ; 1.0,1.52 ]  InitialFluxes=[ 0.8 , -0.8 , 0.7 ]  BreakLoop=off  DiscreteSolver=Trapezoidal iterative  DataType=off  TransfoNumber=1
  Трансформатор_Завод_2_2 : powerlib/Elements/Three-Phase Transformer (Two Windings)  Winding1Connection=Yg  Winding2Connection=Yg  CoreType=Three single-phase transformers  SetSaturation=off  Hysteresis=off  DataFile='hysteresis'  SetInitialFlux=off  Measurements=None  UNITS=pu  NominalPower=[Tr_35_04_Sn_VA, Sys_f_Hz]  Winding1=[Tr_35_04_V_HV_kV*1e3, Tr_35_04_R_pu, Tr_35_04_L_pu]  Winding2=[Tr_35_04_V_LV_kV*1e3, Tr_35_04_R_pu, Tr_35_04_L_pu]  Rm=500  Lm=500  L0=0.5  Saturation=[ 0,0 ; 0.0024,1.2 ; 1.0,1.52 ]  InitialFluxes=[ 0.8 , -0.8 , 0.7 ]  BreakLoop=off  DiscreteSolver=Trapezoidal iterative  DataType=off  TransfoNumber=1
  Трансформатор_Завод_3_1 : powerlib/Elements/Three-Phase Transformer (Two Windings)  Winding1Connection=Yg  Winding2Connection=Yg  CoreType=Three single-phase transformers  SetSaturation=off  Hysteresis=off  DataFile='hysteresis'  SetInitialFlux=off  Measurements=None  UNITS=pu  NominalPower=[Tr_35_04_Sn_VA, Sys_f_Hz]  Winding1=[Tr_35_04_V_HV_kV*1e3, Tr_35_04_R_pu, Tr_35_04_L_pu]  Winding2=[Tr_35_04_V_LV_kV*1e3, Tr_35_04_R_pu, Tr_35_04_L_pu]  Rm=500  Lm=500  L0=0.5  Saturation=[ 0,0 ; 0.0024,1.2 ; 1.0,1.52 ]  InitialFluxes=[ 0.8 , -0.8 , 0.7 ]  BreakLoop=off  DiscreteSolver=Trapezoidal iterative  DataType=off  TransfoNumber=1
  Трансформатор_Завод_3_2 : powerlib/Elements/Three-Phase Transformer (Two Windings)  Winding1Connection=Yg  Winding2Connection=Yg  CoreType=Three single-phase transformers  SetSaturation=off  Hysteresis=off  DataFile='hysteresis'  SetInitialFlux=off  Measurements=None  UNITS=pu  NominalPower=[Tr_35_04_Sn_VA, Sys_f_Hz]  Winding1=[Tr_35_04_V_HV_kV*1e3, Tr_35_04_R_pu, Tr_35_04_L_pu]  Winding2=[Tr_35_04_V_LV_kV*1e3, Tr_35_04_R_pu, Tr_35_04_L_pu]  Rm=500  Lm=500  L0=0.5  Saturation=[ 0,0 ; 0.0024,1.2 ; 1.0,1.52 ]  InitialFluxes=[ 0.8 , -0.8 , 0.7 ]  BreakLoop=off  DiscreteSolver=Trapezoidal iterative  DataType=off  TransfoNumber=1
  Трансформатор_Завод_4_1 : powerlib/Elements/Three-Phase Transformer (Two Windings)  Winding1Connection=Yg  Winding2Connection=Yg  CoreType=Three single-phase transformers  SetSaturation=off  Hysteresis=off  DataFile='hysteresis'  SetInitialFlux=off  Measurements=None  UNITS=pu  NominalPower=[Tr_35_04_Sn_VA, Sys_f_Hz]  Winding1=[Tr_35_04_V_HV_kV*1e3, Tr_35_04_R_pu, Tr_35_04_L_pu]  Winding2=[Tr_35_04_V_LV_kV*1e3, Tr_35_04_R_pu, Tr_35_04_L_pu]  Rm=500  Lm=500  L0=0.5  Saturation=[ 0,0 ; 0.0024,1.2 ; 1.0,1.52 ]  InitialFluxes=[ 0.8 , -0.8 , 0.7 ]  BreakLoop=off  DiscreteSolver=Trapezoidal iterative  DataType=off  TransfoNumber=1
  Трансформатор_Завод_4_2 : powerlib/Elements/Three-Phase Transformer (Two Windings)  Winding1Connection=Yg  Winding2Connection=Yg  CoreType=Three single-phase transformers  SetSaturation=off  Hysteresis=off  DataFile='hysteresis'  SetInitialFlux=off  Measurements=None  UNITS=pu  NominalPower=[Tr_35_04_Sn_VA, Sys_f_Hz]  Winding1=[Tr_35_04_V_HV_kV*1e3, Tr_35_04_R_pu, Tr_35_04_L_pu]  Winding2=[Tr_35_04_V_LV_kV*1e3, Tr_35_04_R_pu, Tr_35_04_L_pu]  Rm=500  Lm=500  L0=0.5  Saturation=[ 0,0 ; 0.0024,1.2 ; 1.0,1.52 ]  InitialFluxes=[ 0.8 , -0.8 , 0.7 ]  BreakLoop=off  DiscreteSolver=Trapezoidal iterative  DataType=off  TransfoNumber=1
  Трансформатор_Завод_5_1 : powerlib/Elements/Three-Phase Transformer (Two Windings)  Winding1Connection=Yg  Winding2Connection=Yg  CoreType=Three single-phase transformers  SetSaturation=off  Hysteresis=off  DataFile='hysteresis'  SetInitialFlux=off  Measurements=None  UNITS=pu  NominalPower=[Tr_35_04_Sn_VA, Sys_f_Hz]  Winding1=[Tr_35_04_V_HV_kV*1e3, Tr_35_04_R_pu, Tr_35_04_L_pu]  Winding2=[Tr_35_04_V_LV_kV*1e3, Tr_35_04_R_pu, Tr_35_04_L_pu]  Rm=500  Lm=500  L0=0.5  Saturation=[ 0,0 ; 0.0024,1.2 ; 1.0,1.52 ]  InitialFluxes=[ 0.8 , -0.8 , 0.7 ]  BreakLoop=off  DiscreteSolver=Trapezoidal iterative  DataType=off  TransfoNumber=1
  Трансформатор_Завод_5_2 : powerlib/Elements/Three-Phase Transformer (Two Windings)  Winding1Connection=Yg  Winding2Connection=Yg  CoreType=Three single-phase transformers  SetSaturation=off  Hysteresis=off  DataFile='hysteresis'  SetInitialFlux=off  Measurements=None  UNITS=pu  NominalPower=[Tr_35_04_Sn_VA, Sys_f_Hz]  Winding1=[Tr_35_04_V_HV_kV*1e3, Tr_35_04_R_pu, Tr_35_04_L_pu]  Winding2=[Tr_35_04_V_LV_kV*1e3, Tr_35_04_R_pu, Tr_35_04_L_pu]  Rm=500  Lm=500  L0=0.5  Saturation=[ 0,0 ; 0.0024,1.2 ; 1.0,1.52 ]  InitialFluxes=[ 0.8 , -0.8 , 0.7 ]  BreakLoop=off  DiscreteSolver=Trapezoidal iterative  DataType=off  TransfoNumber=1
  Трансформатор_Завод_6_1 : powerlib/Elements/Three-Phase Transformer (Two Windings)  Winding1Connection=Yg  Winding2Connection=Yg  CoreType=Three single-phase transformers  SetSaturation=off  Hysteresis=off  DataFile='hysteresis'  SetInitialFlux=off  Measurements=None  UNITS=pu  NominalPower=[Tr_35_04_Sn_VA, Sys_f_Hz]  Winding1=[Tr_35_04_V_HV_kV*1e3, Tr_35_04_R_pu, Tr_35_04_L_pu]  Winding2=[Tr_35_04_V_LV_kV*1e3, Tr_35_04_R_pu, Tr_35_04_L_pu]  Rm=500  Lm=500  L0=0.5  Saturation=[ 0,0 ; 0.0024,1.2 ; 1.0,1.52 ]  InitialFluxes=[ 0.8 , -0.8 , 0.7 ]  BreakLoop=off  DiscreteSolver=Trapezoidal iterative  DataType=off  TransfoNumber=1
  Трансформатор_Завод_6_2 : powerlib/Elements/Three-Phase Transformer (Two Windings)  Winding1Connection=Yg  Winding2Connection=Yg  CoreType=Three single-phase transformers  SetSaturation=off  Hysteresis=off  DataFile='hysteresis'  SetInitialFlux=off  Measurements=None  UNITS=pu  NominalPower=[Tr_35_04_Sn_VA, Sys_f_Hz]  Winding1=[Tr_35_04_V_HV_kV*1e3, Tr_35_04_R_pu, Tr_35_04_L_pu]  Winding2=[Tr_35_04_V_LV_kV*1e3, Tr_35_04_R_pu, Tr_35_04_L_pu]  Rm=500  Lm=500  L0=0.5  Saturation=[ 0,0 ; 0.0024,1.2 ; 1.0,1.52 ]  InitialFluxes=[ 0.8 , -0.8 , 0.7 ]  BreakLoop=off  DiscreteSolver=Trapezoidal iterative  DataType=off  TransfoNumber=1
  Трансформатор_УРП_220_110 : powerlib/Elements/Three-Phase Transformer (Two Windings)  Winding1Connection=Yg  Winding2Connection=Yg  CoreType=Three single-phase transformers  SetSaturation=off  Hysteresis=off  DataFile='hysteresis'  SetInitialFlux=off  Measurements=None  UNITS=pu  NominalPower=[Tr_220_110_Sn_VA, Sys_f_Hz]  Winding1=[Tr_220_110_V_HV_kV*1e3, Tr_220_110_R_pu, Tr_220_110_L_pu]  Winding2=[Tr_220_110_V_LV_kV*1e3, Tr_220_110_R_pu, Tr_220_110_L_pu]  Rm=500  Lm=500  L0=0.5  Saturation=[ 0,0 ; 0.0024,1.2 ; 1.0,1.52 ]  InitialFluxes=[ 0.8 , -0.8 , 0.7 ]  BreakLoop=off  DiscreteSolver=Trapezoidal iterative  DataType=off  TransfoNumber=1
  connections:
  Источник_220кВ/RConn1 -- Магистраль_220кВ/LConn1
  Источник_220кВ/RConn2 -- Магистраль_220кВ/LConn2
  Источник_220кВ/RConn3 -- Магистраль_220кВ/LConn3
  Магистраль_220кВ/RConn1 -- Трансформатор_УРП_220_110/LConn1
  Магистраль_220кВ/RConn2 -- Трансформатор_УРП_220_110/LConn2
  Магистраль_220кВ/RConn3 -- Трансформатор_УРП_220_110/LConn3
  Линия_110кВ_Район_1/LConn1 -- Трансформатор_УРП_220_110/RConn1 -- Линия_110кВ_Район_2/LConn1 -- Линия_110кВ_Район_3/LConn1 -- Линия_110кВ_Район_4/LConn1 -- Линия_110кВ_Район_5/LConn1 -- Линия_110кВ_Район_6/LConn1
  Линия_110кВ_Район_1/LConn2 -- Трансформатор_УРП_220_110/RConn2 -- Линия_110кВ_Район_2/LConn2 -- Линия_110кВ_Район_3/LConn2 -- Линия_110кВ_Район_4/LConn2 -- Линия_110кВ_Район_5/LConn2 -- Линия_110кВ_Район_6/LConn2
  Линия_110кВ_Район_1/LConn3 -- Трансформатор_УРП_220_110/RConn3 -- Линия_110кВ_Район_2/LConn3 -- Линия_110кВ_Район_3/LConn3 -- Линия_110кВ_Район_4/LConn3 -- Линия_110кВ_Район_5/LConn3 -- Линия_110кВ_Район_6/LConn3
  Трансформатор_110_35_Район_1/LConn1 -- Линия_110кВ_Район_1/RConn1 -- Трансформатор_110_6_Район_1/LConn1
  Трансформатор_110_35_Район_1/LConn2 -- Линия_110кВ_Район_1/RConn2 -- Трансформатор_110_6_Район_1/LConn2
  Трансформатор_110_35_Район_1/LConn3 -- Линия_110кВ_Район_1/RConn3 -- Трансформатор_110_6_Район_1/LConn3
  Линия_Завод_1_1/LConn1 -- Трансформатор_110_35_Район_1/RConn1 -- Линия_Завод_1_2/LConn1
  Линия_Завод_1_1/LConn2 -- Трансформатор_110_35_Район_1/RConn2 -- Линия_Завод_1_2/LConn2
  Линия_Завод_1_1/LConn3 -- Трансформатор_110_35_Район_1/RConn3 -- Линия_Завод_1_2/LConn3
  Линия_Завод_1_1/RConn1 -- M_IN_Завод_1_1/LConn1
  Линия_Завод_1_1/RConn2 -- M_IN_Завод_1_1/LConn2
  Линия_Завод_1_1/RConn3 -- M_IN_Завод_1_1/LConn3
  M_IN_Завод_1_1/RConn1 -- Трансформатор_Завод_1_1/LConn1
  M_IN_Завод_1_1/RConn2 -- Трансформатор_Завод_1_1/LConn2
  M_IN_Завод_1_1/RConn3 -- Трансформатор_Завод_1_1/LConn3
  Трансформатор_Завод_1_1/RConn1 -- M_OUT_Завод_1_1/LConn1
  Трансформатор_Завод_1_1/RConn2 -- M_OUT_Завод_1_1/LConn2
  Трансформатор_Завод_1_1/RConn3 -- M_OUT_Завод_1_1/LConn3
  M_OUT_Завод_1_1/RConn1 -- Нагрузка_Завод_1_1/LConn1
  M_OUT_Завод_1_1/RConn2 -- Нагрузка_Завод_1_1/LConn2
  M_OUT_Завод_1_1/RConn3 -- Нагрузка_Завод_1_1/LConn3
  Линия_Завод_1_2/RConn1 -- M_IN_Завод_1_2/LConn1
  Линия_Завод_1_2/RConn2 -- M_IN_Завод_1_2/LConn2
  Линия_Завод_1_2/RConn3 -- M_IN_Завод_1_2/LConn3
  M_IN_Завод_1_2/RConn1 -- Трансформатор_Завод_1_2/LConn1
  M_IN_Завод_1_2/RConn2 -- Трансформатор_Завод_1_2/LConn2
  M_IN_Завод_1_2/RConn3 -- Трансформатор_Завод_1_2/LConn3
  Трансформатор_Завод_1_2/RConn1 -- M_OUT_Завод_1_2/LConn1
  Трансформатор_Завод_1_2/RConn2 -- M_OUT_Завод_1_2/LConn2
  Трансформатор_Завод_1_2/RConn3 -- M_OUT_Завод_1_2/LConn3
  M_OUT_Завод_1_2/RConn1 -- Нагрузка_Завод_1_2/LConn1
  M_OUT_Завод_1_2/RConn2 -- Нагрузка_Завод_1_2/LConn2
  M_OUT_Завод_1_2/RConn3 -- Нагрузка_Завод_1_2/LConn3
  Линия_Город_1_1/LConn1 -- Трансформатор_110_6_Район_1/RConn1 -- Линия_Город_1_2/LConn1 -- Линия_Город_1_3/LConn1 -- Линия_Город_1_4/LConn1
  Линия_Город_1_1/LConn2 -- Трансформатор_110_6_Район_1/RConn2 -- Линия_Город_1_2/LConn2 -- Линия_Город_1_3/LConn2 -- Линия_Город_1_4/LConn2
  Линия_Город_1_1/LConn3 -- Трансформатор_110_6_Район_1/RConn3 -- Линия_Город_1_2/LConn3 -- Линия_Город_1_3/LConn3 -- Линия_Город_1_4/LConn3
  Линия_Город_1_1/RConn1 -- M_IN_Город_1_1/LConn1
  Линия_Город_1_1/RConn2 -- M_IN_Город_1_1/LConn2
  Линия_Город_1_1/RConn3 -- M_IN_Город_1_1/LConn3
  M_IN_Город_1_1/RConn1 -- Трансформатор_Город_1_1/LConn1
  M_IN_Город_1_1/RConn2 -- Трансформатор_Город_1_1/LConn2
  M_IN_Город_1_1/RConn3 -- Трансформатор_Город_1_1/LConn3
  Трансформатор_Город_1_1/RConn1 -- M_OUT_Город_1_1/LConn1
  Трансформатор_Город_1_1/RConn2 -- M_OUT_Город_1_1/LConn2
  Трансформатор_Город_1_1/RConn3 -- M_OUT_Город_1_1/LConn3
  M_OUT_Город_1_1/RConn1 -- Нагрузка_Город_1_1/LConn1
  M_OUT_Город_1_1/RConn2 -- Нагрузка_Город_1_1/LConn2
  M_OUT_Город_1_1/RConn3 -- Нагрузка_Город_1_1/LConn3
  Линия_Город_1_2/RConn1 -- M_IN_Город_1_2/LConn1
  Линия_Город_1_2/RConn2 -- M_IN_Город_1_2/LConn2
  Линия_Город_1_2/RConn3 -- M_IN_Город_1_2/LConn3
  M_IN_Город_1_2/RConn1 -- Трансформатор_Город_1_2/LConn1
  M_IN_Город_1_2/RConn2 -- Трансформатор_Город_1_2/LConn2
  M_IN_Город_1_2/RConn3 -- Трансформатор_Город_1_2/LConn3
  Трансформатор_Город_1_2/RConn1 -- M_OUT_Город_1_2/LConn1
  Трансформатор_Город_1_2/RConn2 -- M_OUT_Город_1_2/LConn2
  Трансформатор_Город_1_2/RConn3 -- M_OUT_Город_1_2/LConn3
  M_OUT_Город_1_2/RConn1 -- Нагрузка_Город_1_2/LConn1
  M_OUT_Город_1_2/RConn2 -- Нагрузка_Город_1_2/LConn2
  M_OUT_Город_1_2/RConn3 -- Нагрузка_Город_1_2/LConn3
  Линия_Город_1_3/RConn1 -- M_IN_Город_1_3/LConn1
  Линия_Город_1_3/RConn2 -- M_IN_Город_1_3/LConn2
  Линия_Город_1_3/RConn3 -- M_IN_Город_1_3/LConn3
  M_IN_Город_1_3/RConn1 -- Трансформатор_Город_1_3/LConn1
  M_IN_Город_1_3/RConn2 -- Трансформатор_Город_1_3/LConn2
  M_IN_Город_1_3/RConn3 -- Трансформатор_Город_1_3/LConn3
  Трансформатор_Город_1_3/RConn1 -- M_OUT_Город_1_3/LConn1
  Трансформатор_Город_1_3/RConn2 -- M_OUT_Город_1_3/LConn2
  Трансформатор_Город_1_3/RConn3 -- M_OUT_Город_1_3/LConn3
  M_OUT_Город_1_3/RConn1 -- Нагрузка_Город_1_3/LConn1
  M_OUT_Город_1_3/RConn2 -- Нагрузка_Город_1_3/LConn2
  M_OUT_Город_1_3/RConn3 -- Нагрузка_Город_1_3/LConn3
  Линия_Город_1_4/RConn1 -- M_IN_Город_1_4/LConn1
  Линия_Город_1_4/RConn2 -- M_IN_Город_1_4/LConn2
  Линия_Город_1_4/RConn3 -- M_IN_Город_1_4/LConn3
  M_IN_Город_1_4/RConn1 -- Трансформатор_Город_1_4/LConn1
  M_IN_Город_1_4/RConn2 -- Трансформатор_Город_1_4/LConn2
  M_IN_Город_1_4/RConn3 -- Трансформатор_Город_1_4/LConn3
  Трансформатор_Город_1_4/RConn1 -- M_OUT_Город_1_4/LConn1
  Трансформатор_Город_1_4/RConn2 -- M_OUT_Город_1_4/LConn2
  Трансформатор_Город_1_4/RConn3 -- M_OUT_Город_1_4/LConn3
  M_OUT_Город_1_4/RConn1 -- Нагрузка_Город_1_4/LConn1
  M_OUT_Город_1_4/RConn2 -- Нагрузка_Город_1_4/LConn2
  M_OUT_Город_1_4/RConn3 -- Нагрузка_Город_1_4/LConn3
  Трансформатор_110_35_Район_2/LConn1 -- Линия_110кВ_Район_2/RConn1 -- Трансформатор_110_6_Район_2/LConn1
  Трансформатор_110_35_Район_2/LConn2 -- Линия_110кВ_Район_2/RConn2 -- Трансформатор_110_6_Район_2/LConn2
  Трансформатор_110_35_Район_2/LConn3 -- Линия_110кВ_Район_2/RConn3 -- Трансформатор_110_6_Район_2/LConn3
  Линия_Завод_2_1/LConn1 -- Трансформатор_110_35_Район_2/RConn1 -- Линия_Завод_2_2/LConn1
  Линия_Завод_2_1/LConn2 -- Трансформатор_110_35_Район_2/RConn2 -- Линия_Завод_2_2/LConn2
  Линия_Завод_2_1/LConn3 -- Трансформатор_110_35_Район_2/RConn3 -- Линия_Завод_2_2/LConn3
  Линия_Завод_2_1/RConn1 -- M_IN_Завод_2_1/LConn1
  Линия_Завод_2_1/RConn2 -- M_IN_Завод_2_1/LConn2
  Линия_Завод_2_1/RConn3 -- M_IN_Завод_2_1/LConn3
  M_IN_Завод_2_1/RConn1 -- Трансформатор_Завод_2_1/LConn1
  M_IN_Завод_2_1/RConn2 -- Трансформатор_Завод_2_1/LConn2
  M_IN_Завод_2_1/RConn3 -- Трансформатор_Завод_2_1/LConn3
  Трансформатор_Завод_2_1/RConn1 -- M_OUT_Завод_2_1/LConn1
  Трансформатор_Завод_2_1/RConn2 -- M_OUT_Завод_2_1/LConn2
  Трансформатор_Завод_2_1/RConn3 -- M_OUT_Завод_2_1/LConn3
  M_OUT_Завод_2_1/RConn1 -- Нагрузка_Завод_2_1/LConn1
  M_OUT_Завод_2_1/RConn2 -- Нагрузка_Завод_2_1/LConn2
  M_OUT_Завод_2_1/RConn3 -- Нагрузка_Завод_2_1/LConn3
  Линия_Завод_2_2/RConn1 -- M_IN_Завод_2_2/LConn1
  Линия_Завод_2_2/RConn2 -- M_IN_Завод_2_2/LConn2
  Линия_Завод_2_2/RConn3 -- M_IN_Завод_2_2/LConn3
  M_IN_Завод_2_2/RConn1 -- Трансформатор_Завод_2_2/LConn1
  M_IN_Завод_2_2/RConn2 -- Трансформатор_Завод_2_2/LConn2
  M_IN_Завод_2_2/RConn3 -- Трансформатор_Завод_2_2/LConn3
  Трансформатор_Завод_2_2/RConn1 -- M_OUT_Завод_2_2/LConn1
  Трансформатор_Завод_2_2/RConn2 -- M_OUT_Завод_2_2/LConn2
  Трансформатор_Завод_2_2/RConn3 -- M_OUT_Завод_2_2/LConn3
  M_OUT_Завод_2_2/RConn1 -- Нагрузка_Завод_2_2/LConn1
  M_OUT_Завод_2_2/RConn2 -- Нагрузка_Завод_2_2/LConn2
  M_OUT_Завод_2_2/RConn3 -- Нагрузка_Завод_2_2/LConn3
  Линия_Город_2_1/LConn1 -- Трансформатор_110_6_Район_2/RConn1 -- Линия_Город_2_2/LConn1 -- Линия_Город_2_3/LConn1 -- Линия_Город_2_4/LConn1
  Линия_Город_2_1/LConn2 -- Трансформатор_110_6_Район_2/RConn2 -- Линия_Город_2_2/LConn2 -- Линия_Город_2_3/LConn2 -- Линия_Город_2_4/LConn2
  Линия_Город_2_1/LConn3 -- Трансформатор_110_6_Район_2/RConn3 -- Линия_Город_2_2/LConn3 -- Линия_Город_2_3/LConn3 -- Линия_Город_2_4/LConn3
  Линия_Город_2_1/RConn1 -- M_IN_Город_2_1/LConn1
  Линия_Город_2_1/RConn2 -- M_IN_Город_2_1/LConn2
  Линия_Город_2_1/RConn3 -- M_IN_Город_2_1/LConn3
  M_IN_Город_2_1/RConn1 -- Трансформатор_Город_2_1/LConn1
  M_IN_Город_2_1/RConn2 -- Трансформатор_Город_2_1/LConn2
  M_IN_Город_2_1/RConn3 -- Трансформатор_Город_2_1/LConn3
  Трансформатор_Город_2_1/RConn1 -- M_OUT_Город_2_1/LConn1
  Трансформатор_Город_2_1/RConn2 -- M_OUT_Город_2_1/LConn2
  Трансформатор_Город_2_1/RConn3 -- M_OUT_Город_2_1/LConn3
  M_OUT_Город_2_1/RConn1 -- Нагрузка_Город_2_1/LConn1
  M_OUT_Город_2_1/RConn2 -- Нагрузка_Город_2_1/LConn2
  M_OUT_Город_2_1/RConn3 -- Нагрузка_Город_2_1/LConn3
  Линия_Город_2_2/RConn1 -- M_IN_Город_2_2/LConn1
  Линия_Город_2_2/RConn2 -- M_IN_Город_2_2/LConn2
  Линия_Город_2_2/RConn3 -- M_IN_Город_2_2/LConn3
  M_IN_Город_2_2/RConn1 -- Трансформатор_Город_2_2/LConn1
  M_IN_Город_2_2/RConn2 -- Трансформатор_Город_2_2/LConn2
  M_IN_Город_2_2/RConn3 -- Трансформатор_Город_2_2/LConn3
  Трансформатор_Город_2_2/RConn1 -- M_OUT_Город_2_2/LConn1
  Трансформатор_Город_2_2/RConn2 -- M_OUT_Город_2_2/LConn2
  Трансформатор_Город_2_2/RConn3 -- M_OUT_Город_2_2/LConn3
  M_OUT_Город_2_2/RConn1 -- Нагрузка_Город_2_2/LConn1
  M_OUT_Город_2_2/RConn2 -- Нагрузка_Город_2_2/LConn2
  M_OUT_Город_2_2/RConn3 -- Нагрузка_Город_2_2/LConn3
  Линия_Город_2_3/RConn1 -- M_IN_Город_2_3/LConn1
  Линия_Город_2_3/RConn2 -- M_IN_Город_2_3/LConn2
  Линия_Город_2_3/RConn3 -- M_IN_Город_2_3/LConn3
  M_IN_Город_2_3/RConn1 -- Трансформатор_Город_2_3/LConn1
  M_IN_Город_2_3/RConn2 -- Трансформатор_Город_2_3/LConn2
  M_IN_Город_2_3/RConn3 -- Трансформатор_Город_2_3/LConn3
  Трансформатор_Город_2_3/RConn1 -- M_OUT_Город_2_3/LConn1
  Трансформатор_Город_2_3/RConn2 -- M_OUT_Город_2_3/LConn2
  Трансформатор_Город_2_3/RConn3 -- M_OUT_Город_2_3/LConn3
  M_OUT_Город_2_3/RConn1 -- Нагрузка_Город_2_3/LConn1
  M_OUT_Город_2_3/RConn2 -- Нагрузка_Город_2_3/LConn2
  M_OUT_Город_2_3/RConn3 -- Нагрузка_Город_2_3/LConn3
  Линия_Город_2_4/RConn1 -- M_IN_Город_2_4/LConn1
  Линия_Город_2_4/RConn2 -- M_IN_Город_2_4/LConn2
  Линия_Город_2_4/RConn3 -- M_IN_Город_2_4/LConn3
  M_IN_Город_2_4/RConn1 -- Трансформатор_Город_2_4/LConn1
  M_IN_Город_2_4/RConn2 -- Трансформатор_Город_2_4/LConn2
  M_IN_Город_2_4/RConn3 -- Трансформатор_Город_2_4/LConn3
  Трансформатор_Город_2_4/RConn1 -- M_OUT_Город_2_4/LConn1
  Трансформатор_Город_2_4/RConn2 -- M_OUT_Город_2_4/LConn2
  Трансформатор_Город_2_4/RConn3 -- M_OUT_Город_2_4/LConn3
  M_OUT_Город_2_4/RConn1 -- Нагрузка_Город_2_4/LConn1
  M_OUT_Город_2_4/RConn2 -- Нагрузка_Город_2_4/LConn2
  M_OUT_Город_2_4/RConn3 -- Нагрузка_Город_2_4/LConn3
  Трансформатор_110_35_Район_3/LConn1 -- Линия_110кВ_Район_3/RConn1 -- Трансформатор_110_6_Район_3/LConn1
  Трансформатор_110_35_Район_3/LConn2 -- Линия_110кВ_Район_3/RConn2 -- Трансформатор_110_6_Район_3/LConn2
  Трансформатор_110_35_Район_3/LConn3 -- Линия_110кВ_Район_3/RConn3 -- Трансформатор_110_6_Район_3/LConn3
  Линия_Завод_3_1/LConn1 -- Трансформатор_110_35_Район_3/RConn1 -- Линия_Завод_3_2/LConn1
  Линия_Завод_3_1/LConn2 -- Трансформатор_110_35_Район_3/RConn2 -- Линия_Завод_3_2/LConn2
  Линия_Завод_3_1/LConn3 -- Трансформатор_110_35_Район_3/RConn3 -- Линия_Завод_3_2/LConn3
  Линия_Завод_3_1/RConn1 -- M_IN_Завод_3_1/LConn1
  Линия_Завод_3_1/RConn2 -- M_IN_Завод_3_1/LConn2
  Линия_Завод_3_1/RConn3 -- M_IN_Завод_3_1/LConn3
  M_IN_Завод_3_1/RConn1 -- Трансформатор_Завод_3_1/LConn1
  M_IN_Завод_3_1/RConn2 -- Трансформатор_Завод_3_1/LConn2
  M_IN_Завод_3_1/RConn3 -- Трансформатор_Завод_3_1/LConn3
  Трансформатор_Завод_3_1/RConn1 -- M_OUT_Завод_3_1/LConn1
  Трансформатор_Завод_3_1/RConn2 -- M_OUT_Завод_3_1/LConn2
  Трансформатор_Завод_3_1/RConn3 -- M_OUT_Завод_3_1/LConn3
  M_OUT_Завод_3_1/RConn1 -- Нагрузка_Завод_3_1/LConn1
  M_OUT_Завод_3_1/RConn2 -- Нагрузка_Завод_3_1/LConn2
  M_OUT_Завод_3_1/RConn3 -- Нагрузка_Завод_3_1/LConn3
  Линия_Завод_3_2/RConn1 -- M_IN_Завод_3_2/LConn1
  Линия_Завод_3_2/RConn2 -- M_IN_Завод_3_2/LConn2
  Линия_Завод_3_2/RConn3 -- M_IN_Завод_3_2/LConn3
  M_IN_Завод_3_2/RConn1 -- Трансформатор_Завод_3_2/LConn1
  M_IN_Завод_3_2/RConn2 -- Трансформатор_Завод_3_2/LConn2
  M_IN_Завод_3_2/RConn3 -- Трансформатор_Завод_3_2/LConn3
  Трансформатор_Завод_3_2/RConn1 -- M_OUT_Завод_3_2/LConn1
  Трансформатор_Завод_3_2/RConn2 -- M_OUT_Завод_3_2/LConn2
  Трансформатор_Завод_3_2/RConn3 -- M_OUT_Завод_3_2/LConn3
  M_OUT_Завод_3_2/RConn1 -- Нагрузка_Завод_3_2/LConn1
  M_OUT_Завод_3_2/RConn2 -- Нагрузка_Завод_3_2/LConn2
  M_OUT_Завод_3_2/RConn3 -- Нагрузка_Завод_3_2/LConn3
  Линия_Город_3_1/LConn1 -- Трансформатор_110_6_Район_3/RConn1 -- Линия_Город_3_2/LConn1 -- Линия_Город_3_3/LConn1 -- Линия_Город_3_4/LConn1
  Линия_Город_3_1/LConn2 -- Трансформатор_110_6_Район_3/RConn2 -- Линия_Город_3_2/LConn2 -- Линия_Город_3_3/LConn2 -- Линия_Город_3_4/LConn2
  Линия_Город_3_1/LConn3 -- Трансформатор_110_6_Район_3/RConn3 -- Линия_Город_3_2/LConn3 -- Линия_Город_3_3/LConn3 -- Линия_Город_3_4/LConn3
  Линия_Город_3_1/RConn1 -- M_IN_Город_3_1/LConn1
  Линия_Город_3_1/RConn2 -- M_IN_Город_3_1/LConn2
  Линия_Город_3_1/RConn3 -- M_IN_Город_3_1/LConn3
  M_IN_Город_3_1/RConn1 -- Трансформатор_Город_3_1/LConn1
  M_IN_Город_3_1/RConn2 -- Трансформатор_Город_3_1/LConn2
  M_IN_Город_3_1/RConn3 -- Трансформатор_Город_3_1/LConn3
  Трансформатор_Город_3_1/RConn1 -- M_OUT_Город_3_1/LConn1
  Трансформатор_Город_3_1/RConn2 -- M_OUT_Город_3_1/LConn2
  Трансформатор_Город_3_1/RConn3 -- M_OUT_Город_3_1/LConn3
  M_OUT_Город_3_1/RConn1 -- Нагрузка_Город_3_1/LConn1
  M_OUT_Город_3_1/RConn2 -- Нагрузка_Город_3_1/LConn2
  M_OUT_Город_3_1/RConn3 -- Нагрузка_Город_3_1/LConn3
  Линия_Город_3_2/RConn1 -- M_IN_Город_3_2/LConn1
  Линия_Город_3_2/RConn2 -- M_IN_Город_3_2/LConn2
  Линия_Город_3_2/RConn3 -- M_IN_Город_3_2/LConn3
  M_IN_Город_3_2/RConn1 -- Трансформатор_Город_3_2/LConn1
  M_IN_Город_3_2/RConn2 -- Трансформатор_Город_3_2/LConn2
  M_IN_Город_3_2/RConn3 -- Трансформатор_Город_3_2/LConn3
  Трансформатор_Город_3_2/RConn1 -- M_OUT_Город_3_2/LConn1
  Трансформатор_Город_3_2/RConn2 -- M_OUT_Город_3_2/LConn2
  Трансформатор_Город_3_2/RConn3 -- M_OUT_Город_3_2/LConn3
  M_OUT_Город_3_2/RConn1 -- Нагрузка_Город_3_2/LConn1
  M_OUT_Город_3_2/RConn2 -- Нагрузка_Город_3_2/LConn2
  M_OUT_Город_3_2/RConn3 -- Нагрузка_Город_3_2/LConn3
  Линия_Город_3_3/RConn1 -- M_IN_Город_3_3/LConn1
  Линия_Город_3_3/RConn2 -- M_IN_Город_3_3/LConn2
  Линия_Город_3_3/RConn3 -- M_IN_Город_3_3/LConn3
  M_IN_Город_3_3/RConn1 -- Трансформатор_Город_3_3/LConn1
  M_IN_Город_3_3/RConn2 -- Трансформатор_Город_3_3/LConn2
  M_IN_Город_3_3/RConn3 -- Трансформатор_Город_3_3/LConn3
  Трансформатор_Город_3_3/RConn1 -- M_OUT_Город_3_3/LConn1
  Трансформатор_Город_3_3/RConn2 -- M_OUT_Город_3_3/LConn2
  Трансформатор_Город_3_3/RConn3 -- M_OUT_Город_3_3/LConn3
  M_OUT_Город_3_3/RConn1 -- Нагрузка_Город_3_3/LConn1
  M_OUT_Город_3_3/RConn2 -- Нагрузка_Город_3_3/LConn2
  M_OUT_Город_3_3/RConn3 -- Нагрузка_Город_3_3/LConn3
  Линия_Город_3_4/RConn1 -- M_IN_Город_3_4/LConn1
  Линия_Город_3_4/RConn2 -- M_IN_Город_3_4/LConn2
  Линия_Город_3_4/RConn3 -- M_IN_Город_3_4/LConn3
  M_IN_Город_3_4/RConn1 -- Трансформатор_Город_3_4/LConn1
  M_IN_Город_3_4/RConn2 -- Трансформатор_Город_3_4/LConn2
  M_IN_Город_3_4/RConn3 -- Трансформатор_Город_3_4/LConn3
  Трансформатор_Город_3_4/RConn1 -- M_OUT_Город_3_4/LConn1
  Трансформатор_Город_3_4/RConn2 -- M_OUT_Город_3_4/LConn2
  Трансформатор_Город_3_4/RConn3 -- M_OUT_Город_3_4/LConn3
  M_OUT_Город_3_4/RConn1 -- Нагрузка_Город_3_4/LConn1
  M_OUT_Город_3_4/RConn2 -- Нагрузка_Город_3_4/LConn2
  M_OUT_Город_3_4/RConn3 -- Нагрузка_Город_3_4/LConn3
  Трансформатор_110_35_Район_4/LConn1 -- Линия_110кВ_Район_4/RConn1 -- Трансформатор_110_6_Район_4/LConn1
  Трансформатор_110_35_Район_4/LConn2 -- Линия_110кВ_Район_4/RConn2 -- Трансформатор_110_6_Район_4/LConn2
  Трансформатор_110_35_Район_4/LConn3 -- Линия_110кВ_Район_4/RConn3 -- Трансформатор_110_6_Район_4/LConn3
  Линия_Завод_4_1/LConn1 -- Трансформатор_110_35_Район_4/RConn1 -- Линия_Завод_4_2/LConn1
  Линия_Завод_4_1/LConn2 -- Трансформатор_110_35_Район_4/RConn2 -- Линия_Завод_4_2/LConn2
  Линия_Завод_4_1/LConn3 -- Трансформатор_110_35_Район_4/RConn3 -- Линия_Завод_4_2/LConn3
  Линия_Завод_4_1/RConn1 -- M_IN_Завод_4_1/LConn1
  Линия_Завод_4_1/RConn2 -- M_IN_Завод_4_1/LConn2
  Линия_Завод_4_1/RConn3 -- M_IN_Завод_4_1/LConn3
  M_IN_Завод_4_1/RConn1 -- Трансформатор_Завод_4_1/LConn1
  M_IN_Завод_4_1/RConn2 -- Трансформатор_Завод_4_1/LConn2
  M_IN_Завод_4_1/RConn3 -- Трансформатор_Завод_4_1/LConn3
  Трансформатор_Завод_4_1/RConn1 -- M_OUT_Завод_4_1/LConn1
  Трансформатор_Завод_4_1/RConn2 -- M_OUT_Завод_4_1/LConn2
  Трансформатор_Завод_4_1/RConn3 -- M_OUT_Завод_4_1/LConn3
  M_OUT_Завод_4_1/RConn1 -- Нагрузка_Завод_4_1/LConn1
  M_OUT_Завод_4_1/RConn2 -- Нагрузка_Завод_4_1/LConn2
  M_OUT_Завод_4_1/RConn3 -- Нагрузка_Завод_4_1/LConn3
  Линия_Завод_4_2/RConn1 -- M_IN_Завод_4_2/LConn1
  Линия_Завод_4_2/RConn2 -- M_IN_Завод_4_2/LConn2
  Линия_Завод_4_2/RConn3 -- M_IN_Завод_4_2/LConn3
  M_IN_Завод_4_2/RConn1 -- Трансформатор_Завод_4_2/LConn1
  M_IN_Завод_4_2/RConn2 -- Трансформатор_Завод_4_2/LConn2
  M_IN_Завод_4_2/RConn3 -- Трансформатор_Завод_4_2/LConn3
  Трансформатор_Завод_4_2/RConn1 -- M_OUT_Завод_4_2/LConn1
  Трансформатор_Завод_4_2/RConn2 -- M_OUT_Завод_4_2/LConn2
  Трансформатор_Завод_4_2/RConn3 -- M_OUT_Завод_4_2/LConn3
  M_OUT_Завод_4_2/RConn1 -- Нагрузка_Завод_4_2/LConn1
  M_OUT_Завод_4_2/RConn2 -- Нагрузка_Завод_4_2/LConn2
  M_OUT_Завод_4_2/RConn3 -- Нагрузка_Завод_4_2/LConn3
  Линия_Город_4_1/LConn1 -- Трансформатор_110_6_Район_4/RConn1 -- Линия_Город_4_2/LConn1 -- Линия_Город_4_3/LConn1 -- Линия_Город_4_4/LConn1
  Линия_Город_4_1/LConn2 -- Трансформатор_110_6_Район_4/RConn2 -- Линия_Город_4_2/LConn2 -- Линия_Город_4_3/LConn2 -- Линия_Город_4_4/LConn2
  Линия_Город_4_1/LConn3 -- Трансформатор_110_6_Район_4/RConn3 -- Линия_Город_4_2/LConn3 -- Линия_Город_4_3/LConn3 -- Линия_Город_4_4/LConn3
  Линия_Город_4_1/RConn1 -- M_IN_Город_4_1/LConn1
  Линия_Город_4_1/RConn2 -- M_IN_Город_4_1/LConn2
  Линия_Город_4_1/RConn3 -- M_IN_Город_4_1/LConn3
  M_IN_Город_4_1/RConn1 -- Трансформатор_Город_4_1/LConn1
  M_IN_Город_4_1/RConn2 -- Трансформатор_Город_4_1/LConn2
  M_IN_Город_4_1/RConn3 -- Трансформатор_Город_4_1/LConn3
  Трансформатор_Город_4_1/RConn1 -- M_OUT_Город_4_1/LConn1
  Трансформатор_Город_4_1/RConn2 -- M_OUT_Город_4_1/LConn2
  Трансформатор_Город_4_1/RConn3 -- M_OUT_Город_4_1/LConn3
  M_OUT_Город_4_1/RConn1 -- Нагрузка_Город_4_1/LConn1
  M_OUT_Город_4_1/RConn2 -- Нагрузка_Город_4_1/LConn2
  M_OUT_Город_4_1/RConn3 -- Нагрузка_Город_4_1/LConn3
  Линия_Город_4_2/RConn1 -- M_IN_Город_4_2/LConn1
  Линия_Город_4_2/RConn2 -- M_IN_Город_4_2/LConn2
  Линия_Город_4_2/RConn3 -- M_IN_Город_4_2/LConn3
  M_IN_Город_4_2/RConn1 -- Трансформатор_Город_4_2/LConn1
  M_IN_Город_4_2/RConn2 -- Трансформатор_Город_4_2/LConn2
  M_IN_Город_4_2/RConn3 -- Трансформатор_Город_4_2/LConn3
  Трансформатор_Город_4_2/RConn1 -- M_OUT_Город_4_2/LConn1
  Трансформатор_Город_4_2/RConn2 -- M_OUT_Город_4_2/LConn2
  Трансформатор_Город_4_2/RConn3 -- M_OUT_Город_4_2/LConn3
  M_OUT_Город_4_2/RConn1 -- Нагрузка_Город_4_2/LConn1
  M_OUT_Город_4_2/RConn2 -- Нагрузка_Город_4_2/LConn2
  M_OUT_Город_4_2/RConn3 -- Нагрузка_Город_4_2/LConn3
  Линия_Город_4_3/RConn1 -- M_IN_Город_4_3/LConn1
  Линия_Город_4_3/RConn2 -- M_IN_Город_4_3/LConn2
  Линия_Город_4_3/RConn3 -- M_IN_Город_4_3/LConn3
  M_IN_Город_4_3/RConn1 -- Трансформатор_Город_4_3/LConn1
  M_IN_Город_4_3/RConn2 -- Трансформатор_Город_4_3/LConn2
  M_IN_Город_4_3/RConn3 -- Трансформатор_Город_4_3/LConn3
  Трансформатор_Город_4_3/RConn1 -- M_OUT_Город_4_3/LConn1
  Трансформатор_Город_4_3/RConn2 -- M_OUT_Город_4_3/LConn2
  Трансформатор_Город_4_3/RConn3 -- M_OUT_Город_4_3/LConn3
  M_OUT_Город_4_3/RConn1 -- Нагрузка_Город_4_3/LConn1
  M_OUT_Город_4_3/RConn2 -- Нагрузка_Город_4_3/LConn2
  M_OUT_Город_4_3/RConn3 -- Нагрузка_Город_4_3/LConn3
  Линия_Город_4_4/RConn1 -- M_IN_Город_4_4/LConn1
  Линия_Город_4_4/RConn2 -- M_IN_Город_4_4/LConn2
  Линия_Город_4_4/RConn3 -- M_IN_Город_4_4/LConn3
  M_IN_Город_4_4/RConn1 -- Трансформатор_Город_4_4/LConn1
  M_IN_Город_4_4/RConn2 -- Трансформатор_Город_4_4/LConn2
  M_IN_Город_4_4/RConn3 -- Трансформатор_Город_4_4/LConn3
  Трансформатор_Город_4_4/RConn1 -- M_OUT_Город_4_4/LConn1
  Трансформатор_Город_4_4/RConn2 -- M_OUT_Город_4_4/LConn2
  Трансформатор_Город_4_4/RConn3 -- M_OUT_Город_4_4/LConn3
  M_OUT_Город_4_4/RConn1 -- Нагрузка_Город_4_4/LConn1
  M_OUT_Город_4_4/RConn2 -- Нагрузка_Город_4_4/LConn2
  M_OUT_Город_4_4/RConn3 -- Нагрузка_Город_4_4/LConn3
  Трансформатор_110_35_Район_5/LConn1 -- Линия_110кВ_Район_5/RConn1 -- Трансформатор_110_6_Район_5/LConn1
  Трансформатор_110_35_Район_5/LConn2 -- Линия_110кВ_Район_5/RConn2 -- Трансформатор_110_6_Район_5/LConn2
  Трансформатор_110_35_Район_5/LConn3 -- Линия_110кВ_Район_5/RConn3 -- Трансформатор_110_6_Район_5/LConn3
  Линия_Завод_5_1/LConn1 -- Трансформатор_110_35_Район_5/RConn1 -- Линия_Завод_5_2/LConn1
  Линия_Завод_5_1/LConn2 -- Трансформатор_110_35_Район_5/RConn2 -- Линия_Завод_5_2/LConn2
  Линия_Завод_5_1/LConn3 -- Трансформатор_110_35_Район_5/RConn3 -- Линия_Завод_5_2/LConn3
  Линия_Завод_5_1/RConn1 -- M_IN_Завод_5_1/LConn1
  Линия_Завод_5_1/RConn2 -- M_IN_Завод_5_1/LConn2
  Линия_Завод_5_1/RConn3 -- M_IN_Завод_5_1/LConn3
  M_IN_Завод_5_1/RConn1 -- Трансформатор_Завод_5_1/LConn1
  M_IN_Завод_5_1/RConn2 -- Трансформатор_Завод_5_1/LConn2
  M_IN_Завод_5_1/RConn3 -- Трансформатор_Завод_5_1/LConn3
  Трансформатор_Завод_5_1/RConn1 -- M_OUT_Завод_5_1/LConn1
  Трансформатор_Завод_5_1/RConn2 -- M_OUT_Завод_5_1/LConn2
  Трансформатор_Завод_5_1/RConn3 -- M_OUT_Завод_5_1/LConn3
  M_OUT_Завод_5_1/RConn1 -- Нагрузка_Завод_5_1/LConn1
  M_OUT_Завод_5_1/RConn2 -- Нагрузка_Завод_5_1/LConn2
  M_OUT_Завод_5_1/RConn3 -- Нагрузка_Завод_5_1/LConn3
  Линия_Завод_5_2/RConn1 -- M_IN_Завод_5_2/LConn1
  Линия_Завод_5_2/RConn2 -- M_IN_Завод_5_2/LConn2
  Линия_Завод_5_2/RConn3 -- M_IN_Завод_5_2/LConn3
  M_IN_Завод_5_2/RConn1 -- Трансформатор_Завод_5_2/LConn1
  M_IN_Завод_5_2/RConn2 -- Трансформатор_Завод_5_2/LConn2
  M_IN_Завод_5_2/RConn3 -- Трансформатор_Завод_5_2/LConn3
  Трансформатор_Завод_5_2/RConn1 -- M_OUT_Завод_5_2/LConn1
  Трансформатор_Завод_5_2/RConn2 -- M_OUT_Завод_5_2/LConn2
  Трансформатор_Завод_5_2/RConn3 -- M_OUT_Завод_5_2/LConn3
  M_OUT_Завод_5_2/RConn1 -- Нагрузка_Завод_5_2/LConn1
  M_OUT_Завод_5_2/RConn2 -- Нагрузка_Завод_5_2/LConn2
  M_OUT_Завод_5_2/RConn3 -- Нагрузка_Завод_5_2/LConn3
  Линия_Город_5_1/LConn1 -- Трансформатор_110_6_Район_5/RConn1 -- Линия_Город_5_2/LConn1 -- Линия_Город_5_3/LConn1 -- Линия_Город_5_4/LConn1
  Линия_Город_5_1/LConn2 -- Трансформатор_110_6_Район_5/RConn2 -- Линия_Город_5_2/LConn2 -- Линия_Город_5_3/LConn2 -- Линия_Город_5_4/LConn2
  Линия_Город_5_1/LConn3 -- Трансформатор_110_6_Район_5/RConn3 -- Линия_Город_5_2/LConn3 -- Линия_Город_5_3/LConn3 -- Линия_Город_5_4/LConn3
  Линия_Город_5_1/RConn1 -- M_IN_Город_5_1/LConn1
  Линия_Город_5_1/RConn2 -- M_IN_Город_5_1/LConn2
  Линия_Город_5_1/RConn3 -- M_IN_Город_5_1/LConn3
  M_IN_Город_5_1/RConn1 -- Трансформатор_Город_5_1/LConn1
  M_IN_Город_5_1/RConn2 -- Трансформатор_Город_5_1/LConn2
  M_IN_Город_5_1/RConn3 -- Трансформатор_Город_5_1/LConn3
  Трансформатор_Город_5_1/RConn1 -- M_OUT_Город_5_1/LConn1
  Трансформатор_Город_5_1/RConn2 -- M_OUT_Город_5_1/LConn2
  Трансформатор_Город_5_1/RConn3 -- M_OUT_Город_5_1/LConn3
  M_OUT_Город_5_1/RConn1 -- Нагрузка_Город_5_1/LConn1
  M_OUT_Город_5_1/RConn2 -- Нагрузка_Город_5_1/LConn2
  M_OUT_Город_5_1/RConn3 -- Нагрузка_Город_5_1/LConn3
  Линия_Город_5_2/RConn1 -- M_IN_Город_5_2/LConn1
  Линия_Город_5_2/RConn2 -- M_IN_Город_5_2/LConn2
  Линия_Город_5_2/RConn3 -- M_IN_Город_5_2/LConn3
  M_IN_Город_5_2/RConn1 -- Трансформатор_Город_5_2/LConn1
  M_IN_Город_5_2/RConn2 -- Трансформатор_Город_5_2/LConn2
  M_IN_Город_5_2/RConn3 -- Трансформатор_Город_5_2/LConn3
  Трансформатор_Город_5_2/RConn1 -- M_OUT_Город_5_2/LConn1
  Трансформатор_Город_5_2/RConn2 -- M_OUT_Город_5_2/LConn2
  Трансформатор_Город_5_2/RConn3 -- M_OUT_Город_5_2/LConn3
  M_OUT_Город_5_2/RConn1 -- Нагрузка_Город_5_2/LConn1
  M_OUT_Город_5_2/RConn2 -- Нагрузка_Город_5_2/LConn2
  M_OUT_Город_5_2/RConn3 -- Нагрузка_Город_5_2/LConn3
  Линия_Город_5_3/RConn1 -- M_IN_Город_5_3/LConn1
  Линия_Город_5_3/RConn2 -- M_IN_Город_5_3/LConn2
  Линия_Город_5_3/RConn3 -- M_IN_Город_5_3/LConn3
  M_IN_Город_5_3/RConn1 -- Трансформатор_Город_5_3/LConn1
  M_IN_Город_5_3/RConn2 -- Трансформатор_Город_5_3/LConn2
  M_IN_Город_5_3/RConn3 -- Трансформатор_Город_5_3/LConn3
  Трансформатор_Город_5_3/RConn1 -- M_OUT_Город_5_3/LConn1
  Трансформатор_Город_5_3/RConn2 -- M_OUT_Город_5_3/LConn2
  Трансформатор_Город_5_3/RConn3 -- M_OUT_Город_5_3/LConn3
  M_OUT_Город_5_3/RConn1 -- Нагрузка_Город_5_3/LConn1
  M_OUT_Город_5_3/RConn2 -- Нагрузка_Город_5_3/LConn2
  M_OUT_Город_5_3/RConn3 -- Нагрузка_Город_5_3/LConn3
  Линия_Город_5_4/RConn1 -- M_IN_Город_5_4/LConn1
  Линия_Город_5_4/RConn2 -- M_IN_Город_5_4/LConn2
  Линия_Город_5_4/RConn3 -- M_IN_Город_5_4/LConn3
  M_IN_Город_5_4/RConn1 -- Трансформатор_Город_5_4/LConn1
  M_IN_Город_5_4/RConn2 -- Трансформатор_Город_5_4/LConn2
  M_IN_Город_5_4/RConn3 -- Трансформатор_Город_5_4/LConn3
  Трансформатор_Город_5_4/RConn1 -- M_OUT_Город_5_4/LConn1
  Трансформатор_Город_5_4/RConn2 -- M_OUT_Город_5_4/LConn2
  Трансформатор_Город_5_4/RConn3 -- M_OUT_Город_5_4/LConn3
  M_OUT_Город_5_4/RConn1 -- Нагрузка_Город_5_4/LConn1
  M_OUT_Город_5_4/RConn2 -- Нагрузка_Город_5_4/LConn2
  M_OUT_Город_5_4/RConn3 -- Нагрузка_Город_5_4/LConn3
  Трансформатор_110_35_Район_6/LConn1 -- Линия_110кВ_Район_6/RConn1 -- Трансформатор_110_6_Район_6/LConn1
  Трансформатор_110_35_Район_6/LConn2 -- Линия_110кВ_Район_6/RConn2 -- Трансформатор_110_6_Район_6/LConn2
  Трансформатор_110_35_Район_6/LConn3 -- Линия_110кВ_Район_6/RConn3 -- Трансформатор_110_6_Район_6/LConn3
  Трансформатор_110_35_Район_6/RConn1 -- Линия_Завод_6_1/LConn1
  Трансформатор_110_35_Район_6/RConn2 -- Линия_Завод_6_1/LConn2
  Трансформатор_110_35_Район_6/RConn3 -- Линия_Завод_6_1/LConn3
  M_IN_Завод_6_1/LConn1 -- Линия_Завод_6_1/RConn1 -- Линия_Завод_6_2/LConn1
  M_IN_Завод_6_1/LConn2 -- Линия_Завод_6_1/RConn2 -- Линия_Завод_6_2/LConn2
  M_IN_Завод_6_1/LConn3 -- Линия_Завод_6_1/RConn3 -- Линия_Завод_6_2/LConn3
  M_IN_Завод_6_1/RConn1 -- Трансформатор_Завод_6_1/LConn1
  M_IN_Завод_6_1/RConn2 -- Трансформатор_Завод_6_1/LConn2
  M_IN_Завод_6_1/RConn3 -- Трансформатор_Завод_6_1/LConn3
  Трансформатор_Завод_6_1/RConn1 -- M_OUT_Завод_6_1/LConn1
  Трансформатор_Завод_6_1/RConn2 -- M_OUT_Завод_6_1/LConn2
  Трансформатор_Завод_6_1/RConn3 -- M_OUT_Завод_6_1/LConn3
  M_OUT_Завод_6_1/RConn1 -- Нагрузка_Завод_6_1/LConn1
  M_OUT_Завод_6_1/RConn2 -- Нагрузка_Завод_6_1/LConn2
  M_OUT_Завод_6_1/RConn3 -- Нагрузка_Завод_6_1/LConn3
  Линия_Завод_6_2/RConn1 -- M_IN_Завод_6_2/LConn1
  Линия_Завод_6_2/RConn2 -- M_IN_Завод_6_2/LConn2
  Линия_Завод_6_2/RConn3 -- M_IN_Завод_6_2/LConn3
  M_IN_Завод_6_2/RConn1 -- Трансформатор_Завод_6_2/LConn1
  M_IN_Завод_6_2/RConn2 -- Трансформатор_Завод_6_2/LConn2
  M_IN_Завод_6_2/RConn3 -- Трансформатор_Завод_6_2/LConn3
  Трансформатор_Завод_6_2/RConn1 -- M_OUT_Завод_6_2/LConn1
  Трансформатор_Завод_6_2/RConn2 -- M_OUT_Завод_6_2/LConn2
  Трансформатор_Завод_6_2/RConn3 -- M_OUT_Завод_6_2/LConn3
  M_OUT_Завод_6_2/RConn1 -- Нагрузка_Завод_6_2/LConn1
  M_OUT_Завод_6_2/RConn2 -- Нагрузка_Завод_6_2/LConn2
  M_OUT_Завод_6_2/RConn3 -- Нагрузка_Завод_6_2/LConn3
  Трансформатор_110_6_Район_6/RConn1 -- Линия_Город_6_1/LConn1
  Трансформатор_110_6_Район_6/RConn2 -- Линия_Город_6_1/LConn2
  Трансформатор_110_6_Район_6/RConn3 -- Линия_Город_6_1/LConn3
  M_IN_Город_6_1/LConn1 -- Линия_Город_6_1/RConn1 -- Линия_Город_6_2/LConn1
  M_IN_Город_6_1/LConn2 -- Линия_Город_6_1/RConn2 -- Линия_Город_6_2/LConn2
  M_IN_Город_6_1/LConn3 -- Линия_Город_6_1/RConn3 -- Линия_Город_6_2/LConn3
  M_IN_Город_6_1/RConn1 -- Трансформатор_Город_6_1/LConn1
  M_IN_Город_6_1/RConn2 -- Трансформатор_Город_6_1/LConn2
  M_IN_Город_6_1/RConn3 -- Трансформатор_Город_6_1/LConn3
  Трансформатор_Город_6_1/RConn1 -- M_OUT_Город_6_1/LConn1
  Трансформатор_Город_6_1/RConn2 -- M_OUT_Город_6_1/LConn2
  Трансформатор_Город_6_1/RConn3 -- M_OUT_Город_6_1/LConn3
  M_OUT_Город_6_1/RConn1 -- Нагрузка_Город_6_1/LConn1
  M_OUT_Город_6_1/RConn2 -- Нагрузка_Город_6_1/LConn2
  M_OUT_Город_6_1/RConn3 -- Нагрузка_Город_6_1/LConn3
  M_IN_Город_6_2/LConn1 -- Линия_Город_6_2/RConn1 -- Линия_Город_6_3/LConn1
  M_IN_Город_6_2/LConn2 -- Линия_Город_6_2/RConn2 -- Линия_Город_6_3/LConn2
  M_IN_Город_6_2/LConn3 -- Линия_Город_6_2/RConn3 -- Линия_Город_6_3/LConn3
  M_IN_Город_6_2/RConn1 -- Трансформатор_Город_6_2/LConn1
  M_IN_Город_6_2/RConn2 -- Трансформатор_Город_6_2/LConn2
  M_IN_Город_6_2/RConn3 -- Трансформатор_Город_6_2/LConn3
  Трансформатор_Город_6_2/RConn1 -- M_OUT_Город_6_2/LConn1
  Трансформатор_Город_6_2/RConn2 -- M_OUT_Город_6_2/LConn2
  Трансформатор_Город_6_2/RConn3 -- M_OUT_Город_6_2/LConn3
  M_OUT_Город_6_2/RConn1 -- Нагрузка_Город_6_2/LConn1
  M_OUT_Город_6_2/RConn2 -- Нагрузка_Город_6_2/LConn2
  M_OUT_Город_6_2/RConn3 -- Нагрузка_Город_6_2/LConn3
  M_IN_Город_6_3/LConn1 -- Линия_Город_6_3/RConn1 -- Линия_Город_6_4/LConn1
  M_IN_Город_6_3/LConn2 -- Линия_Город_6_3/RConn2 -- Линия_Город_6_4/LConn2
  M_IN_Город_6_3/LConn3 -- Линия_Город_6_3/RConn3 -- Линия_Город_6_4/LConn3
  M_IN_Город_6_3/RConn1 -- Трансформатор_Город_6_3/LConn1
  M_IN_Город_6_3/RConn2 -- Трансформатор_Город_6_3/LConn2
  M_IN_Город_6_3/RConn3 -- Трансформатор_Город_6_3/LConn3
  Трансформатор_Город_6_3/RConn1 -- M_OUT_Город_6_3/LConn1
  Трансформатор_Город_6_3/RConn2 -- M_OUT_Город_6_3/LConn2
  Трансформатор_Город_6_3/RConn3 -- M_OUT_Город_6_3/LConn3
  M_OUT_Город_6_3/RConn1 -- Нагрузка_Город_6_3/LConn1
  M_OUT_Город_6_3/RConn2 -- Нагрузка_Город_6_3/LConn2
  M_OUT_Город_6_3/RConn3 -- Нагрузка_Город_6_3/LConn3
  Линия_Город_6_4/RConn1 -- M_IN_Город_6_4/LConn1
  Линия_Город_6_4/RConn2 -- M_IN_Город_6_4/LConn2
  Линия_Город_6_4/RConn3 -- M_IN_Город_6_4/LConn3
  M_IN_Город_6_4/RConn1 -- Трансформатор_Город_6_4/LConn1
  M_IN_Город_6_4/RConn2 -- Трансформатор_Город_6_4/LConn2
  M_IN_Город_6_4/RConn3 -- Трансформатор_Город_6_4/LConn3
  Трансформатор_Город_6_4/RConn1 -- M_OUT_Город_6_4/LConn1
  Трансформатор_Город_6_4/RConn2 -- M_OUT_Город_6_4/LConn2
  Трансформатор_Город_6_4/RConn3 -- M_OUT_Город_6_4/LConn3
  M_OUT_Город_6_4/RConn1 -- Нагрузка_Город_6_4/LConn1
  M_OUT_Город_6_4/RConn2 -- Нагрузка_Город_6_4/LConn2
  M_OUT_Город_6_4/RConn3 -- Нагрузка_Город_6_4/LConn3
